simulink library "xbsIndex_r4"  (Simulink 7.1)
(part 7 of 9)

      mask init:
      | try
      |   tmp_gcb = gcb;
      |   tmp_gcbh = gcbh;
      |   if (strcmp('SysGenIndex',get_param(bdroot(tmp_gcbh),'tag')) && ~isempty(regexp(bdroot(tmp_gcb), '^xbs', 'once')))
      |     return;
      |   end;
      |   xlMungeMaskParams;
      |   block_config = 'sysgen:coregenimport_config';
      | 
      |   block_type='rs_decoder_v8_0';
      | 
      |   serialized_declarations = '{''aclken''=>''Bool'',''aresetn''=>''Bool'',''code_specification''=>''String'',''data_symbols''=>''Int'',''define_supported_r_in_values''=>''Bool'',''dsptool_ready''=>''Bool'',''erase''=>''Bool'',''error_statistics''=>''Bool'',''field_polynomial''=>''Int'',''generator_start''=>''Int'',''info''=>''Bool'',''ip_name''=>''String'',''ip_version''=>''String'',''ipcore_do_not_force_period''=>''Bool'',''ipcore_usecache''=>''Bool'',''ipcore_useipmodelcache''=>''Bool'',''marker_bits''=>''Bool'',''memory_style''=>''String'',''number_of_channels''=>''Int'',''number_of_marker_bits''=>''Int'',''number_of_puncture_patterns''=>''Int'',''number_of_supported_r_in_values''=>''Int'',''original_delayed_data''=>''Bool'',''output_check_symbols''=>''Bool'',''port_translation_map''=>''String'',''puncture_definition_file''=>''String'',''scaling_factor''=>''Int'',''self_recovering''=>''Bool'',''structural_sim''=>''Bool'',''supported_r_in_definition_file''=>''String'',''symbol_width''=>''String'',''symbols_per_block''=>''Int'',''trim_axipin_name''=>''Int'',''variable_block_length''=>''Bool'',''variable_number_of_check_symbols''=>''Bool'',''wrapper_available''=>''Bool'',''block_type''=>''String''}';
      |   ptable_ = xlblockprep(get_param(tmp_gcb, 'MaskWSVariables'));
      |   try
      |     xlBlockMoveCallback(tmp_gcbh);
      |   catch 
      |      clear global xl_updateicon_recursion_guard;
      |   end;
      | catch
      |   global dbgsysgen;
      |   if(~isempty(dbgsysgen) && dbgsysgen)
      |     e = regexprep(lasterr, '\n', '\nError: ');
      |     disp(['Error: While running MaskInit code on block ' tmp_gcb ': ' e]);
      |     error(e);
      |   end
      | end
      settings: CopyFcn=xlBlockMoveCallback(gcbh);  DeleteFcn=xlDestroyGui(gcbh);  ModelCloseFcn=xlDestroyGui(gcbh);  PreSaveFcn=xlBlockPreSaveCallback(gcbh);  PostSaveFcn=xlBlockPostSaveCallback(gcbh);  DestroyFcn=xlDestroyGui(gcbh);  OpenFcn=xlOpenGui(gcbh, 'rs_decoder_v8_0_gui.xml', @rs_decoder_v8_0_enablement, @rs_decoder_v8_0_action)  CloseFcn=xlDestroyGui(gcbh);  MoveFcn=xlBlockMoveCallback(gcbh);
      mask Help: eval('');xlDoc('-book','sysgen','-topic','Reed_Solomon_Decoder_8_0');
      mask StyleString: popup(Custom|DVB|ATSC|G.709|CCSDS|IESS-308(All)|IESS-308(126)|IESS-308(194)|IESS-308(208)|IESS-308(219)|IESS-308(225)|IEEE-802.16),popup(3|4|5|6|7|8|9|10|11|12),edit,edit,edit,edit,checkbox,edit,edit,edit,checkbox,edit,checkbox,edit,edit,edit,checkbox,popup(Automatic|Block|Distributed),edit,checkbox,edit,edit,edit,checkbox,edit,checkbox,edit,checkbox,edit,checkbox,edit,checkbox,edit,checkbox,edit,checkbox,edit,checkbox,edit,edit,edit,edit,edit,edit,edit,edit,edit,edit,edit,edit,edit,edit,edit,edit,edit
      mask Display:
      | fprintf('','COMMENT: begin icon graphics');
      | patch([0 0 2 2 ],[142 60 60 142 ],[5.650000e-001 6.550000e-001 5.500000e-001 ]);
      | patch([0 0 2 2 ],[52 30 30 52 ],[4.100000e-001 4.700000e-001 4.000000e-001 ]);
      | patch([0 0 2 2 ],[22 0 0 22 ],[2.550000e-001 2.850000e-001 2.500000e-001 ]);
      | patch([93 93 95 95 ],[125 117 117 125 ],[5.650000e-001 6.550000e-001 5.500000e-001 ]);
      | patch([93 93 95 95 ],[115 87 87 115 ],[4.100000e-001 4.700000e-001 4.000000e-001 ]);
      | patch([93 93 95 95 ],[85 47 47 85 ],[2.550000e-001 2.850000e-001 2.500000e-001 ]);
      | patch([93 93 95 95 ],[45 17 17 45 ],[7.200000e-001 8.400000e-001 7.000000e-001 ]);
      | patch([2 92 92 2 2 ],[0 0 142 142 0 ],[7.200000e-001 8.400000e-001 7.000000e-001 ]);
      | plot([2 92 92 2 2 ],[0 0 142 142 0 ]);
      | 
      | 
      | patch([18.075 36.86 49.86 62.86 75.86 49.86 31.075 18.075 ],[85.43 85.43 98.43 85.43 98.43 98.43 98.43 85.43 ],[1 1 1 ]);
      | patch([31.075 49.86 36.86 18.075 31.075 ],[72.43 72.43 85.43 85.43 72.43 ],[0.916 0.952 0.91 ]);
      | patch([18.075 36.86 49.86 31.075 18.075 ],[59.43 59.43 72.43 72.43 59.43 ],[1 1 1 ]);
      | patch([31.075 75.86 62.86 49.86 36.86 18.075 31.075 ],[46.43 46.43 59.43 46.43 59.43 59.43 46.43 ],[0.916 0.952 0.91 ]);
      | fprintf('','COMMENT: end icon graphics');
      | fprintf('','COMMENT: begin icon text');
      | color('black');port_label('input',1,'  input_tvalid  ');
      | color('black');port_label('input',2,'  input_tdata_data_in  ');
      | color('black');port_label('input',3,'  input_tlast  ');
      | color('black');port_label('input',4,'  output_tready  ');
      | color('black');port_label('input',5,'  stat_tready  ');
      | color('black');port_label('output',1,'  input_tready  ');
      | color('black');port_label('output',2,'  output_tvalid  ');
      | color('black');port_label('output',3,'  output_tdata_data_out  ');
      | color('black');port_label('output',4,'  output_tlast  ');
      | color('black');port_label('output',5,'  stat_tvalid  ');
      | color('black');port_label('output',6,'  stat_tdata_err_cnt  ');
      | color('black');port_label('output',7,'  stat_tdata_err_found  ');
      | color('black');port_label('output',8,'  stat_tdata_fail  ');
      | color('black');port_label('output',9,'  event_s_input_tlast_missing  ');
      | color('black');port_label('output',10,'  event_s_input_tlast_unexpected  ');
      | color('black');port_label('output',11,'  event_s_ctrl_tdata_invalid  ');
      | fprintf('','COMMENT: end icon text');
  "Reed-Solomon Encoder 6.1 " : S-Function  LoadFcn=xlBlockLoadCallback(gcbh);  FunctionName=sysgen  Parameters=ptable_  EnableBusSupport=off  mask(Xilinx Reed-Solomon Encoder 6.1 Block){infoedit=Reed-Solomon Encoder 6.1. The encoder transforms each block of k information symbols presented serially at the input port to a block of n symbols presented serially at the output port., code_specification_sgadvanced=, code_specification=Custom, number_of_channels=1, variable_number_of_check_symbols_sgadvanced=, variable_number_of_check_symbols=off, variable_block_length_sgadvanced=, variable_block_length=off, nd_sgadvanced=, nd=off, rdy_sgadvanced=, rdy=off, rfd_sgadvanced=, rfd=off, rffd_sgadvanced=, rffd=off, rst_sgadvanced=, rst=off, en_sgadvanced=, en=off, symbol_width_sgadvanced=, symbol_width=8, symbol_per_block=255, data_symbols=239, field_polynomial=0, generator_start=0, scaling_factor=1, memory_style_sgadvanced=, memory_style=Automatic, check_symbol_generator_sgadvanced=, check_symbol_generator=Fixed_Architecture, xl_use_area_sgadvanced=, xl_use_area=off, xl_area=[0,0,0,0,0,0,0], ip_name=Reed-Solomon Encoder, ip_version=6.1, has_advanced_control=0, sggui_pos=-1,-1,-1,-1, block_type=rs_encoder_v6_1, block_version=, sg_icon_stat=95,142,-1,-1,white,green,0,07734,right,,[ ],[ ], sg_mask_display=|, sg_list_contents=, sg_blockgui_xml=}
      mask sg_mask_display=|
      | fprintf('','COMMENT: begin icon graphics');
      | patch([0 95 95 0 0 ],[0 0 142 142 0 ],[0.72 0.84 0.7 ]);
      | plot([0 95 95 0 0 ],[0 0 142 142 0 ]);
      | patch([18.075 36.86 49.86 62.86 75.86 49.86 31.075 18.075 ],[85.43 85.43 98.43 85.43 98.43 98.43 98.43 85.43 ],[1 1 1 ]);
      | patch([31.075 49.86 36.86 18.075 31.075 ],[72.43 72.43 85.43 85.43 72.43 ],[0.916 0.952 0.91 ]);
      | patch([18.075 36.86 49.86 31.075 18.075 ],[59.43 59.43 72.43 72.43 59.43 ],[1 1 1 ]);
      | patch([31.075 75.86 62.86 49.86 36.86 18.075 31.075 ],[46.43 46.43 59.43 46.43 59.43 59.43 46.43 ],[0.916 0.952 0.91 ]);
      | fprintf('','COMMENT: end icon graphics');
      | fprintf('','COMMENT: begin icon text');
      | fprintf('','COMMENT: end icon text');
      mask prompts: infoedit ""; code_specification_sgadvanced ""; code_specification "Code specification (Predefined settings for popular standards)"; number_of_channels "Number of channels (Symbols for each channel are interlaced on DATA_IN and DATA_OUT)"; variable_number_of_check_symbols_sgadvanced ""; variable_number_of_check_symbols "Variable number of check symbols (Adds R_IN port)"; variable_block_length_sgadvanced ""; variable_block_length "Variable block length (Adds N_IN port)"; nd_sgadvanced ""; rdy_sgadvanced ""; rfd_sgadvanced ""; rffd_sgadvanced ""; rst_sgadvanced ""; en_sgadvanced ""; symbol_width_sgadvanced ""; symbol_width "Symbol width (Bus width of DATA_IN and DATA_OUT)"; symbol_per_block "Symbol per block (Total number of symbols in an encoded block, including check symbols)"; data_symbols "Data symbols (Number of original information symbols in block, prior to encoding)"; field_polynomial "Field polynomial (Galois Field primitive polynomial (enter in decimal))"; generator_start "Generator start (Galois Field logarithm of the first root of the Generator Polynomial)"; scaling_factor "Scaling factor (Scaling factor for Generator Polynomial root index)"; memory_style_sgadvanced ""; memory_style "Memory style (Force core to use this style of internal memory. 'Automatic' means let core decide)"; check_symbol_generator_sgadvanced ""; check_symbol_generator "Check symbol generator (Fixed architecture cannot be optimized)"; xl_use_area_sgadvanced ""; xl_use_area "Define FPGA area for resource estimation"; xl_area "FPGA area [slices, FFs, BRAMs, LUTs, IOBs, emb. mults, TBUFs]"; ip_name ""; ip_version ""; has_advanced_control ""; sggui_pos ""; block_type ""; block_version ""; sg_icon_stat ""; sg_mask_display ""; sg_list_contents ""; sg_blockgui_xml ""
      mask help: Reed-Solomon Encoder 6.1. The encoder transforms each block of k information symbols presented serially at the input port to a block of n symbols presented serially at the output port.
      mask init:
      | try
      |   tmp_gcb = gcb;
      |   tmp_gcbh = gcbh;
      |   if (strcmp('SysGenIndex',get_param(bdroot(tmp_gcbh),'tag')) && ~isempty(regexp(bdroot(tmp_gcb), '^xbs', 'once')))
      |     return;
      |   end;
      |   xlMungeMaskParams;
      |   block_config = 'sysgen_blockset:Removed_config';
      | 
      |   block_type='rs_encoder_v6_1';
      | nport = get_param(gcbh, 'ports');
      | nin = nport(1);
      | nout = nport(2);
      | 
      |   serialized_declarations = '{''check_symbol_generator''=>''String'',''code_specification''=>''String'',''data_symbols''=>''Int'',''en''=>''Bool'',''field_polynomial''=>''Int'',''generator_start''=>''Int'',''ip_name''=>''String'',''ip_version''=>''String'',''memory_style''=>''String'',''nd''=>''Bool'',''number_of_channels''=>''Int'',''rdy''=>''Bool'',''rfd''=>''Bool'',''rffd''=>''Bool'',''rst''=>''Bool'',''scaling_factor''=>''Int'',''symbol_per_block''=>''Int'',''symbol_width''=>''String'',''variable_block_length''=>''Bool'',''variable_number_of_check_symbols''=>''Bool'',''xl_use_area''=>''Bool'',''block_type''=>''String'',''nin''=>''Double'',''nout''=>''Double''}';
      |   ptable_ = xlblockprep(get_param(tmp_gcb, 'MaskWSVariables'));
      |   try
      |     xlBlockMoveCallback(tmp_gcbh);
      |   catch 
      |      clear global xl_updateicon_recursion_guard;
      |   end;
      | catch
      |   global dbgsysgen;
      |   if(~isempty(dbgsysgen) && dbgsysgen)
      |     e = regexprep(lasterr, '\n', '\nError: ');
      |     disp(['Error: While running MaskInit code on block ' tmp_gcb ': ' e]);
      |     error(e);
      |   end
      | end
      settings: CopyFcn=xlBlockMoveCallback(gcbh);  DeleteFcn=xlDestroyGui(gcbh);  ModelCloseFcn=xlDestroyGui(gcbh);  PreSaveFcn=xlBlockPreSaveCallback(gcbh);  PostSaveFcn=xlBlockPostSaveCallback(gcbh);  DestroyFcn=xlDestroyGui(gcbh);  OpenFcn=xlOpenGui(gcbh, 'rs_encoder_v6_1_gui.xml', @xlremovedenablement, -1)  CloseFcn=xlDestroyGui(gcbh);  MoveFcn=xlBlockMoveCallback(gcbh);
      mask Help: eval('');xlDoc('-book','sysgen','-topic','Reed_Solomon_Encoder_6_1');
      mask StyleString: edit,edit,popup(Custom|DVB|ATSC|CCSDS|ITU_J_83_Annex_B|IESS_308_126|IESS_308_194|IESS_308_208|IESS_308_219|IESS_308_225),edit,edit,checkbox,edit,checkbox,edit,checkbox,edit,checkbox,edit,checkbox,edit,checkbox,edit,checkbox,edit,checkbox,edit,popup(3|4|5|6|7|8|9|10|11|12),edit,edit,edit,edit,edit,edit,popup(Automatic|Block|Distributed),edit,popup(Fixed_Architecture|Optimized_For_Area|Optimized_For_Flexibility),edit,checkbox,edit,edit,edit,edit,edit,edit,edit,edit,edit,edit,edit
      mask Display:
      | fprintf('','COMMENT: begin icon graphics');
      | patch([0 95 95 0 0 ],[0 0 142 142 0 ],[0.72 0.84 0.7 ]);
      | plot([0 95 95 0 0 ],[0 0 142 142 0 ]);
      | patch([18.075 36.86 49.86 62.86 75.86 49.86 31.075 18.075 ],[85.43 85.43 98.43 85.43 98.43 98.43 98.43 85.43 ],[1 1 1 ]);
      | patch([31.075 49.86 36.86 18.075 31.075 ],[72.43 72.43 85.43 85.43 72.43 ],[0.916 0.952 0.91 ]);
      | patch([18.075 36.86 49.86 31.075 18.075 ],[59.43 59.43 72.43 72.43 59.43 ],[1 1 1 ]);
      | patch([31.075 75.86 62.86 49.86 36.86 18.075 31.075 ],[46.43 46.43 59.43 46.43 59.43 59.43 46.43 ],[0.916 0.952 0.91 ]);
      | fprintf('','COMMENT: end icon graphics');
      | fprintf('','COMMENT: begin icon text');
      | fprintf('','COMMENT: end icon text');
  "Reed-Solomon Encoder 7.0 " : S-Function  LoadFcn=xlBlockLoadCallback(gcbh);  FunctionName=sysgen  Parameters=ptable_  EnableBusSupport=off  mask(Xilinx Reed-Solomon Encoder 7.0  Block){code_specification=Custom, variable_number_of_check_symbols_sgadvanced=, variable_number_of_check_symbols=off, variable_block_length_sgadvanced=, variable_block_length=off, symbol_width=8, field_polynomial=0, scaling_factor=1, generator_start=0, symbol_per_block=255, data_symbols=239, check_symbol_generator_sgadvanced=, check_symbol_generator=Fixed_Architecture, memory_style=Automatic, number_of_channels=1, ce_sgadvanced=, ce=off, rdy_sgadvanced=, rdy=off, nd_sgadvanced=, nd=off, rfd_sgadvanced=, rfd=off, sclr_sgadvanced=, sclr=off, rffd_sgadvanced=, rffd=off, ip_name=Reed-Solomon Encoder, ip_version=7.0, dsptool_ready=false, ipcore_usecache=true, ipcore_useipmodelcache=true, wrapper_available=true, port_translation_map={ 'ce' => 'en', 'sclr' => 'rst'}, structural_sim=true, ipcore_do_not_force_period=true, has_advanced_control=0, sggui_pos=-1,-1,-1,-1, block_type=rs_encoder_v7_0, block_version=, sg_icon_stat=95,142,3,2,white,green,0,abcad2e4,right,,[ ],[ ], sg_mask_display=|, sg_list_contents=, sg_blockgui_xml=}
      mask sg_mask_display=|
      | fprintf('','COMMENT: begin icon graphics');
      | patch([0 95 95 0 0 ],[0 0 142 142 0 ],[0.72 0.84 0.7 ]);
      | plot([0 95 95 0 0 ],[0 0 142 142 0 ]);
      | patch([18.075 36.86 49.86 62.86 75.86 49.86 31.075 18.075 ],[85.43 85.43 98.43 85.43 98.43 98.43 98.43 85.43 ],[1 1 1 ]);
      | patch([31.075 49.86 36.86 18.075 31.075 ],[72.43 72.43 85.43 85.43 72.43 ],[0.916 0.952 0.91 ]);
      | patch([18.075 36.86 49.86 31.075 18.075 ],[59.43 59.43 72.43 72.43 59.43 ],[1 1 1 ]);
      | patch([31.075 75.86 62.86 49.86 36.86 18.075 31.075 ],[46.43 46.43 59.43 46.43 59.43 59.43 46.43 ],[0.916 0.952 0.91 ]);
      | fprintf('','COMMENT: end icon graphics');
      | fprintf('','COMMENT: begin icon text');
      | color('black');port_label('input',1,'data_in');
      | color('black');port_label('input',2,'bypass');
      | color('black');port_label('input',3,'start');
      | color('black');port_label('output',1,'data_out');
      | color('black');port_label('output',2,'info');
      | fprintf('','COMMENT: end icon text');
      mask prompts: code_specification "Code Specification"; variable_number_of_check_symbols_sgadvanced ""; variable_number_of_check_symbols "Variable Number Of Check Symbols (r)"; variable_block_length_sgadvanced ""; variable_block_length "Variable Block Length"; symbol_width "Symbol Width"; field_polynomial "Field Polynomial"; scaling_factor "Scaling Factor (h)"; generator_start "Generator Start"; symbol_per_block "Symbols Per Block (n)"; data_symbols "Data Symbols (k)"; check_symbol_generator_sgadvanced ""; check_symbol_generator ""; memory_style "Memory Style"; number_of_channels "Number Of Channels"; ce_sgadvanced ""; rdy_sgadvanced ""; nd_sgadvanced ""; rfd_sgadvanced ""; sclr_sgadvanced ""; rffd_sgadvanced ""; ip_name ""; ip_version ""; dsptool_ready ""; ipcore_usecache ""; ipcore_useipmodelcache ""; wrapper_available ""; port_translation_map ""; structural_sim ""; ipcore_do_not_force_period ""; has_advanced_control ""; sggui_pos ""; block_type ""; block_version ""; sg_icon_stat ""; sg_mask_display ""; sg_list_contents ""; sg_blockgui_xml ""
      mask help: Xilinx Reed-Solomon Encoder 7.0
      mask init:
      | try
      |   tmp_gcb = gcb;
      |   tmp_gcbh = gcbh;
      |   if (strcmp('SysGenIndex',get_param(bdroot(tmp_gcbh),'tag')) && ~isempty(regexp(bdroot(tmp_gcb), '^xbs', 'once')))
      |     return;
      |   end;
      |   xlMungeMaskParams;
      |   block_config = 'sysgen:coregenimport_config';
      | 
      |   block_type='rs_encoder_v7_0';
      | 
      |   serialized_declarations = '{''ce''=>''Bool'',''check_symbol_generator''=>''String'',''code_specification''=>''String'',''data_symbols''=>''Int'',''dsptool_ready''=>''Bool'',''field_polynomial''=>''Int'',''generator_start''=>''Int'',''ip_name''=>''String'',''ip_version''=>''String'',''ipcore_do_not_force_period''=>''Bool'',''ipcore_usecache''=>''Bool'',''ipcore_useipmodelcache''=>''Bool'',''memory_style''=>''String'',''nd''=>''Bool'',''number_of_channels''=>''Int'',''port_translation_map''=>''String'',''rdy''=>''Bool'',''rfd''=>''Bool'',''rffd''=>''Bool'',''scaling_factor''=>''Int'',''sclr''=>''Bool'',''structural_sim''=>''Bool'',''symbol_per_block''=>''Int'',''symbol_width''=>''String'',''variable_block_length''=>''Bool'',''variable_number_of_check_symbols''=>''Bool'',''wrapper_available''=>''Bool'',''block_type''=>''String''}';
      |   ptable_ = xlblockprep(get_param(tmp_gcb, 'MaskWSVariables'));
      |   try
      |     xlBlockMoveCallback(tmp_gcbh);
      |   catch 
      |      clear global xl_updateicon_recursion_guard;
      |   end;
      | catch
      |   global dbgsysgen;
      |   if(~isempty(dbgsysgen) && dbgsysgen)
      |     e = regexprep(lasterr, '\n', '\nError: ');
      |     disp(['Error: While running MaskInit code on block ' tmp_gcb ': ' e]);
      |     error(e);
      |   end
      | end
      settings: CopyFcn=xlBlockMoveCallback(gcbh);  DeleteFcn=xlDestroyGui(gcbh);  ModelCloseFcn=xlDestroyGui(gcbh);  PreSaveFcn=xlBlockPreSaveCallback(gcbh);  PostSaveFcn=xlBlockPostSaveCallback(gcbh);  DestroyFcn=xlDestroyGui(gcbh);  OpenFcn=xlOpenGui(gcbh, 'rs_encoder_v7_0_gui.xml', @xlipmagiccallback_pass_evaluate_params, @xlipmagicaction)  CloseFcn=xlDestroyGui(gcbh);  MoveFcn=xlBlockMoveCallback(gcbh);
      mask Help: eval('');xlDoc('-book','sysgen','-topic','Reed_Solomon_Encoder_7_0');
      mask StyleString: popup(Custom|DVB|ATSC|G_709|ETSI_BRAN|CCSDS|ITU_J_83_Annex_B|IESS_308_126|IESS_308_194|IESS_308_208|IESS_308_219|IESS_308_225),edit,checkbox,edit,checkbox,popup(3|4|5|6|7|8|9|10|11|12),edit,edit,edit,edit,edit,edit,popup(Fixed_Architecture|Optimized_For_Area|Optimized_For_Flexibility),popup(Automatic|Block|Distributed),edit,edit,checkbox,edit,checkbox,edit,checkbox,edit,checkbox,edit,checkbox,edit,checkbox,edit,edit,edit,edit,edit,edit,edit,edit,edit,edit,edit,edit,edit,edit,edit,edit,edit
      mask Display:
      | fprintf('','COMMENT: begin icon graphics');
      | patch([0 95 95 0 0 ],[0 0 142 142 0 ],[0.72 0.84 0.7 ]);
      | plot([0 95 95 0 0 ],[0 0 142 142 0 ]);
      | patch([18.075 36.86 49.86 62.86 75.86 49.86 31.075 18.075 ],[85.43 85.43 98.43 85.43 98.43 98.43 98.43 85.43 ],[1 1 1 ]);
      | patch([31.075 49.86 36.86 18.075 31.075 ],[72.43 72.43 85.43 85.43 72.43 ],[0.916 0.952 0.91 ]);
      | patch([18.075 36.86 49.86 31.075 18.075 ],[59.43 59.43 72.43 72.43 59.43 ],[1 1 1 ]);
      | patch([31.075 75.86 62.86 49.86 36.86 18.075 31.075 ],[46.43 46.43 59.43 46.43 59.43 59.43 46.43 ],[0.916 0.952 0.91 ]);
      | fprintf('','COMMENT: end icon graphics');
      | fprintf('','COMMENT: begin icon text');
      | color('black');port_label('input',1,'data_in');
      | color('black');port_label('input',2,'bypass');
      | color('black');port_label('input',3,'start');
      | color('black');port_label('output',1,'data_out');
      | color('black');port_label('output',2,'info');
      | fprintf('','COMMENT: end icon text');
  "Reed-Solomon Encoder 7.1 " : S-Function  LoadFcn=xlBlockLoadCallback(gcbh);  FunctionName=sysgen  Parameters=ptable_  EnableBusSupport=off  mask(Xilinx Reed-Solomon Encoder 7.1  Block){code_specification=Custom, variable_number_of_check_symbols_sgadvanced=, variable_number_of_check_symbols=off, variable_block_length_sgadvanced=, variable_block_length=off, symbol_width=8, field_polynomial=0, scaling_factor=1, generator_start=0, symbol_per_block=255, data_symbols=239, check_symbol_generator_sgadvanced=, check_symbol_generator=Fixed_Architecture, memory_style=Automatic, number_of_channels=1, ce_sgadvanced=, ce=off, rdy_sgadvanced=, rdy=off, nd_sgadvanced=, nd=off, rfd_sgadvanced=, rfd=off, sclr_sgadvanced=, sclr=off, rffd_sgadvanced=, rffd=off, ip_name=Reed-Solomon Encoder, ip_version=7.1, dsptool_ready=false, ipcore_usecache=true, ipcore_useipmodelcache=true, wrapper_available=true, port_translation_map={ 'ce' => 'en', 'sclr' => 'rst'}, structural_sim=false, ipcore_do_not_force_period=true, has_advanced_control=0, sggui_pos=-1,-1,-1,-1, block_type=rs_encoder_v7_1, block_version=, sg_icon_stat=95,142,3,2,white,green,0,abcad2e4,right,,[ ],[ ], sg_mask_display=|, sg_list_contents=, sg_blockgui_xml=}
      mask sg_mask_display=|
      | fprintf('','COMMENT: begin icon graphics');
      | patch([0 95 95 0 0 ],[0 0 142 142 0 ],[0.72 0.84 0.7 ]);
      | plot([0 95 95 0 0 ],[0 0 142 142 0 ]);
      | patch([18.075 36.86 49.86 62.86 75.86 49.86 31.075 18.075 ],[85.43 85.43 98.43 85.43 98.43 98.43 98.43 85.43 ],[1 1 1 ]);
      | patch([31.075 49.86 36.86 18.075 31.075 ],[72.43 72.43 85.43 85.43 72.43 ],[0.916 0.952 0.91 ]);
      | patch([18.075 36.86 49.86 31.075 18.075 ],[59.43 59.43 72.43 72.43 59.43 ],[1 1 1 ]);
      | patch([31.075 75.86 62.86 49.86 36.86 18.075 31.075 ],[46.43 46.43 59.43 46.43 59.43 59.43 46.43 ],[0.916 0.952 0.91 ]);
      | fprintf('','COMMENT: end icon graphics');
      | fprintf('','COMMENT: begin icon text');
      | color('black');port_label('input',1,'data_in');
      | color('black');port_label('input',2,'bypass');
      | color('black');port_label('input',3,'start');
      | color('black');port_label('output',1,'data_out');
      | color('black');port_label('output',2,'info');
      | fprintf('','COMMENT: end icon text');
      mask prompts: code_specification "Code Specification"; variable_number_of_check_symbols_sgadvanced ""; variable_number_of_check_symbols "Variable Number Of Check Symbols (r)"; variable_block_length_sgadvanced ""; variable_block_length "Variable Block Length"; symbol_width "Symbol Width"; field_polynomial "Field Polynomial"; scaling_factor "Scaling Factor (h)"; generator_start "Generator Start"; symbol_per_block "Symbols Per Block (n)"; data_symbols "Data Symbols (k)"; check_symbol_generator_sgadvanced ""; check_symbol_generator ""; memory_style "Memory Style"; number_of_channels "Number Of Channels"; ce_sgadvanced ""; rdy_sgadvanced ""; nd_sgadvanced ""; rfd_sgadvanced ""; sclr_sgadvanced ""; rffd_sgadvanced ""; ip_name ""; ip_version ""; dsptool_ready ""; ipcore_usecache ""; ipcore_useipmodelcache ""; wrapper_available ""; port_translation_map ""; structural_sim ""; ipcore_do_not_force_period ""; has_advanced_control ""; sggui_pos ""; block_type ""; block_version ""; sg_icon_stat ""; sg_mask_display ""; sg_list_contents ""; sg_blockgui_xml ""
      mask help: Xilinx Reed-Solomon Encoder 7.1
      mask init:
      | try
      |   tmp_gcb = gcb;
      |   tmp_gcbh = gcbh;
      |   if (strcmp('SysGenIndex',get_param(bdroot(tmp_gcbh),'tag')) && ~isempty(regexp(bdroot(tmp_gcb), '^xbs', 'once')))
      |     return;
      |   end;
      |   xlMungeMaskParams;
      |   block_config = 'sysgen:coregenimport_config';
      | 
      |   block_type='rs_encoder_v7_1';
      | 
      |   serialized_declarations = '{''ce''=>''Bool'',''check_symbol_generator''=>''String'',''code_specification''=>''String'',''data_symbols''=>''Int'',''dsptool_ready''=>''Bool'',''field_polynomial''=>''Int'',''generator_start''=>''Int'',''ip_name''=>''String'',''ip_version''=>''String'',''ipcore_do_not_force_period''=>''Bool'',''ipcore_usecache''=>''Bool'',''ipcore_useipmodelcache''=>''Bool'',''memory_style''=>''String'',''nd''=>''Bool'',''number_of_channels''=>''Int'',''port_translation_map''=>''String'',''rdy''=>''Bool'',''rfd''=>''Bool'',''rffd''=>''Bool'',''scaling_factor''=>''Int'',''sclr''=>''Bool'',''structural_sim''=>''Bool'',''symbol_per_block''=>''Int'',''symbol_width''=>''String'',''variable_block_length''=>''Bool'',''variable_number_of_check_symbols''=>''Bool'',''wrapper_available''=>''Bool'',''block_type''=>''String''}';
      |   ptable_ = xlblockprep(get_param(tmp_gcb, 'MaskWSVariables'));
      |   try
      |     xlBlockMoveCallback(tmp_gcbh);
      |   catch 
      |      clear global xl_updateicon_recursion_guard;
      |   end;
      | catch
      |   global dbgsysgen;
      |   if(~isempty(dbgsysgen) && dbgsysgen)
      |     e = regexprep(lasterr, '\n', '\nError: ');
      |     disp(['Error: While running MaskInit code on block ' tmp_gcb ': ' e]);
      |     error(e);
      |   end
      | end
      settings: CopyFcn=xlBlockMoveCallback(gcbh);  DeleteFcn=xlDestroyGui(gcbh);  ModelCloseFcn=xlDestroyGui(gcbh);  PreSaveFcn=xlBlockPreSaveCallback(gcbh);  PostSaveFcn=xlBlockPostSaveCallback(gcbh);  DestroyFcn=xlDestroyGui(gcbh);  OpenFcn=xlOpenGui(gcbh, 'rs_encoder_v7_1_gui.xml', @xlipmagiccallback_pass_evaluate_params, @xlipmagicaction)  CloseFcn=xlDestroyGui(gcbh);  MoveFcn=xlBlockMoveCallback(gcbh);
      mask Help: eval('');xlDoc('-book','sysgen','-topic','Reed_Solomon_Encoder_7_1');
      mask StyleString: popup(Custom|DVB|ATSC|G_709|ETSI_BRAN|CCSDS|ITU_J_83_Annex_B|IESS_308_126|IESS_308_194|IESS_308_208|IESS_308_219|IESS_308_225),edit,checkbox,edit,checkbox,popup(3|4|5|6|7|8|9|10|11|12),edit,edit,edit,edit,edit,edit,popup(Fixed_Architecture|Optimized_For_Area|Optimized_For_Flexibility),popup(Automatic|Block|Distributed),edit,edit,checkbox,edit,checkbox,edit,checkbox,edit,checkbox,edit,checkbox,edit,checkbox,edit,edit,edit,edit,edit,edit,edit,edit,edit,edit,edit,edit,edit,edit,edit,edit,edit
      mask Display:
      | fprintf('','COMMENT: begin icon graphics');
      | patch([0 95 95 0 0 ],[0 0 142 142 0 ],[0.72 0.84 0.7 ]);
      | plot([0 95 95 0 0 ],[0 0 142 142 0 ]);
      | patch([18.075 36.86 49.86 62.86 75.86 49.86 31.075 18.075 ],[85.43 85.43 98.43 85.43 98.43 98.43 98.43 85.43 ],[1 1 1 ]);
      | patch([31.075 49.86 36.86 18.075 31.075 ],[72.43 72.43 85.43 85.43 72.43 ],[0.916 0.952 0.91 ]);
      | patch([18.075 36.86 49.86 31.075 18.075 ],[59.43 59.43 72.43 72.43 59.43 ],[1 1 1 ]);
      | patch([31.075 75.86 62.86 49.86 36.86 18.075 31.075 ],[46.43 46.43 59.43 46.43 59.43 59.43 46.43 ],[0.916 0.952 0.91 ]);
      | fprintf('','COMMENT: end icon graphics');
      | fprintf('','COMMENT: begin icon text');
      | color('black');port_label('input',1,'data_in');
      | color('black');port_label('input',2,'bypass');
      | color('black');port_label('input',3,'start');
      | color('black');port_label('output',1,'data_out');
      | color('black');port_label('output',2,'info');
      | fprintf('','COMMENT: end icon text');
  "Reed-Solomon Encoder 8.0 " : S-Function  LoadFcn=xlBlockLoadCallback(gcbh);  FunctionName=sysgen  Parameters=ptable_  EnableBusSupport=off  mask(Xilinx Reed-Solomon Encoder 8.0  Block){code_specification=Custom, variable_number_of_check_symbols_sgadvanced=, variable_number_of_check_symbols=off, variable_block_length_sgadvanced=, variable_block_length=off, symbol_width=8, field_polynomial=0, scaling_factor=1, generator_start=0, symbol_per_block=255, data_symbols=239, check_symbol_generator_sgadvanced=, check_symbol_generator=Fixed_Architecture, memory_style=Automatic, number_of_channels=1, aclken_sgadvanced=, aclken=off, output_has_tready_sgadvanced=, output_has_tready=off, aresetn_sgadvanced=, aresetn=off, info_sgadvanced=, info=off, marker_bits_sgadvanced=, marker_bits=off, number_of_marker_bits=1, trim_axipin_name=on, ip_name=Reed-Solomon Encoder, ip_version=8.0, dsptool_ready=false, ipcore_usecache=true, ipcore_useipmodelcache=true, wrapper_available=true, port_translation_map={ 'aclken' => 'en', 'aresetn' => 'rst'}, structural_sim=false, ipcore_do_not_force_period=true, has_advanced_control=0, sggui_pos=-1,-1,-1,-1, block_type=rs_encoder_v8_0, block_version=, sg_icon_stat=215,223,3,6,white,green,0,414e65fd,right,,[2 2 2 ],[2 3 3 3 1 1 ], sg_mask_display=|, sg_list_contents=, sg_blockgui_xml=}
      mask sg_mask_display=|
      | fprintf('','COMMENT: begin icon graphics');
      | patch([0 0 4 4 ],[210 8 8 210 ],[5.133333e-001 5.933333e-001 5.000000e-001 ]);
      | patch([211 211 215 215 ],[211 187 187 211 ],[5.133333e-001 5.933333e-001 5.000000e-001 ]);
      | patch([211 211 215 215 ],[176 82 82 176 ],[3.066667e-001 3.466667e-001 3.000000e-001 ]);
      | patch([211 211 215 215 ],[71 12 12 71 ],[7.200000e-001 8.400000e-001 7.000000e-001 ]);
      | patch([4 210 210 4 4 ],[0 0 223 223 0 ],[7.200000e-001 8.400000e-001 7.000000e-001 ]);
      | plot([4 210 210 4 4 ],[0 0 223 223 0 ]);
      |
      |
      | patch([40.25 83.6 113.6 143.6 173.6 113.6 70.25 40.25 ],[144.3 144.3 174.3 144.3 174.3 174.3 174.3 144.3 ],[1 1 1 ]);
      | patch([70.25 113.6 83.6 40.25 70.25 ],[114.3 114.3 144.3 144.3 114.3 ],[0.916 0.952 0.91 ]);
      | patch([40.25 83.6 113.6 70.25 40.25 ],[84.3 84.3 114.3 114.3 84.3 ],[1 1 1 ]);
      | patch([70.25 173.6 143.6 113.6 83.6 40.25 70.25 ],[54.3 54.3 84.3 54.3 84.3 84.3 54.3 ],[0.916 0.952 0.91 ]);
      | fprintf('','COMMENT: end icon graphics');
      | fprintf('','COMMENT: begin icon text');
      | color('black');port_label('input',1,'  input_tvalid  ');
      | color('black');port_label('input',2,'  input_tdata_data_in  ');
      | color('black');port_label('input',3,'  input_tlast  ');
      | color('black');port_label('output',1,'  input_tready  ');
      | color('black');port_label('output',2,'  output_tvalid  ');
      | color('black');port_label('output',3,'  output_tdata_data_out  ');
      | color('black');port_label('output',4,'  output_tlast  ');
      | color('black');port_label('output',5,'  event_s_input_tlast_missing  ');
      | color('black');port_label('output',6,'  event_s_input_tlast_unexpected  ');
      | fprintf('','COMMENT: end icon text');
      mask prompts: code_specification "Code Specification"; variable_number_of_check_symbols_sgadvanced ""; variable_number_of_check_symbols "Variable Number Of Check Symbols (r)"; variable_block_length_sgadvanced ""; variable_block_length "Variable Block Length"; symbol_width "Symbol Width"; field_polynomial "Field Polynomial"; scaling_factor "Scaling Factor (h)"; generator_start "Generator Start"; symbol_per_block "Symbols Per Block (n)"; data_symbols "Data Symbols (k)"; check_symbol_generator_sgadvanced ""; check_symbol_generator ""; memory_style "Memory Style"; number_of_channels "Number Of Channels"; aclken_sgadvanced ""; output_has_tready_sgadvanced ""; output_has_tready "Output TREADY"; aresetn_sgadvanced ""; info_sgadvanced ""; info "Info bit"; marker_bits_sgadvanced ""; marker_bits "Marker Bits"; number_of_marker_bits "Number Of Marker Bits"; trim_axipin_name "Display shortened port names"; ip_name ""; ip_version ""; dsptool_ready ""; ipcore_usecache ""; ipcore_useipmodelcache ""; wrapper_available ""; port_translation_map ""; structural_sim ""; ipcore_do_not_force_period ""; has_advanced_control ""; sggui_pos ""; block_type ""; block_version ""; sg_icon_stat ""; sg_mask_display ""; sg_list_contents ""; sg_blockgui_xml ""
      mask help: Xilinx Reed-Solomon Encoder 8.0
      mask init:
      | try
      |   tmp_gcb = gcb;
      |   tmp_gcbh = gcbh;
      |   if (strcmp('SysGenIndex',get_param(bdroot(tmp_gcbh),'tag')) && ~isempty(regexp(bdroot(tmp_gcb), '^xbs', 'once')))
      |     return;
      |   end;
      |   xlMungeMaskParams;
      |   block_config = 'sysgen:coregenimport_config';
      | 
      |   block_type='rs_encoder_v8_0';
      | 
      |   serialized_declarations = '{''aclken''=>''Bool'',''aresetn''=>''Bool'',''check_symbol_generator''=>''String'',''code_specification''=>''String'',''data_symbols''=>''Int'',''dsptool_ready''=>''Bool'',''field_polynomial''=>''Int'',''generator_start''=>''Int'',''info''=>''Bool'',''ip_name''=>''String'',''ip_version''=>''String'',''ipcore_do_not_force_period''=>''Bool'',''ipcore_usecache''=>''Bool'',''ipcore_useipmodelcache''=>''Bool'',''marker_bits''=>''Bool'',''memory_style''=>''String'',''number_of_channels''=>''Int'',''number_of_marker_bits''=>''Int'',''output_has_tready''=>''Bool'',''port_translation_map''=>''String'',''scaling_factor''=>''Int'',''structural_sim''=>''Bool'',''symbol_per_block''=>''Int'',''symbol_width''=>''String'',''trim_axipin_name''=>''Int'',''variable_block_length''=>''Bool'',''variable_number_of_check_symbols''=>''Bool'',''wrapper_available''=>''Bool'',''block_type''=>''String''}';
      |   ptable_ = xlblockprep(get_param(tmp_gcb, 'MaskWSVariables'));
      |   try
      |     xlBlockMoveCallback(tmp_gcbh);
      |   catch 
      |      clear global xl_updateicon_recursion_guard;
      |   end;
      | catch
      |   global dbgsysgen;
      |   if(~isempty(dbgsysgen) && dbgsysgen)
      |     e = regexprep(lasterr, '\n', '\nError: ');
      |     disp(['Error: While running MaskInit code on block ' tmp_gcb ': ' e]);
      |     error(e);
      |   end
      | end
      settings: CopyFcn=xlBlockMoveCallback(gcbh);  DeleteFcn=xlDestroyGui(gcbh);  ModelCloseFcn=xlDestroyGui(gcbh);  PreSaveFcn=xlBlockPreSaveCallback(gcbh);  PostSaveFcn=xlBlockPostSaveCallback(gcbh);  DestroyFcn=xlDestroyGui(gcbh);  OpenFcn=xlOpenGui(gcbh, 'rs_encoder_v8_0_gui.xml', @xlipmagiccallback_pass_evaluate_params, @xlipmagicaction)  CloseFcn=xlDestroyGui(gcbh);  MoveFcn=xlBlockMoveCallback(gcbh);
      mask Help: eval('');xlDoc('-book','sysgen','-topic','Reed_Solomon_Encoder_8_0');
      mask StyleString: popup(Custom|DVB|ATSC|G_709|ETSI_BRAN|CCSDS|ITU_J_83_Annex_B|IESS_308_126|IESS_308_194|IESS_308_208|IESS_308_219|IESS_308_225),edit,checkbox,edit,checkbox,popup(3|4|5|6|7|8|9|10|11|12),edit,edit,edit,edit,edit,edit,popup(Fixed_Architecture|Optimized_For_Area|Optimized_For_Flexibility),popup(Automatic|Block|Distributed),edit,edit,checkbox,edit,checkbox,edit,checkbox,edit,checkbox,edit,checkbox,edit,checkbox,edit,edit,edit,edit,edit,edit,edit,edit,edit,edit,edit,edit,edit,edit,edit,edit,edit
      mask Display:
      | fprintf('','COMMENT: begin icon graphics');
      | patch([0 0 4 4 ],[210 8 8 210 ],[5.133333e-001 5.933333e-001 5.000000e-001 ]);
      | patch([211 211 215 215 ],[211 187 187 211 ],[5.133333e-001 5.933333e-001 5.000000e-001 ]);
      | patch([211 211 215 215 ],[176 82 82 176 ],[3.066667e-001 3.466667e-001 3.000000e-001 ]);
      | patch([211 211 215 215 ],[71 12 12 71 ],[7.200000e-001 8.400000e-001 7.000000e-001 ]);
      | patch([4 210 210 4 4 ],[0 0 223 223 0 ],[7.200000e-001 8.400000e-001 7.000000e-001 ]);
      | plot([4 210 210 4 4 ],[0 0 223 223 0 ]);
      | 
      | 
      | patch([40.25 83.6 113.6 143.6 173.6 113.6 70.25 40.25 ],[144.3 144.3 174.3 144.3 174.3 174.3 174.3 144.3 ],[1 1 1 ]);
      | patch([70.25 113.6 83.6 40.25 70.25 ],[114.3 114.3 144.3 144.3 114.3 ],[0.916 0.952 0.91 ]);
      | patch([40.25 83.6 113.6 70.25 40.25 ],[84.3 84.3 114.3 114.3 84.3 ],[1 1 1 ]);
      | patch([70.25 173.6 143.6 113.6 83.6 40.25 70.25 ],[54.3 54.3 84.3 54.3 84.3 84.3 54.3 ],[0.916 0.952 0.91 ]);
      | fprintf('','COMMENT: end icon graphics');
      | fprintf('','COMMENT: begin icon text');
      | color('black');port_label('input',1,'  input_tvalid  ');
      | color('black');port_label('input',2,'  input_tdata_data_in  ');
      | color('black');port_label('input',3,'  input_tlast  ');
      | color('black');port_label('output',1,'  input_tready  ');
      | color('black');port_label('output',2,'  output_tvalid  ');
      | color('black');port_label('output',3,'  output_tdata_data_out  ');
      | color('black');port_label('output',4,'  output_tlast  ');
      | color('black');port_label('output',5,'  event_s_input_tlast_missing  ');
      | color('black');port_label('output',6,'  event_s_input_tlast_unexpected  ');
      | fprintf('','COMMENT: end icon text');
  Register : S-Function  LoadFcn=xlBlockLoadCallback(gcbh);  FunctionName=sysgen  Parameters=ptable_  EnableBusSupport=off  mask(Xilinx Register Block){init=0, rst_sgadvanced=, rst=off, en_sgadvanced=, en=off, dbl_ovrd_sgadvanced=, dbl_ovrd=off, xl_use_area_sgadvanced=, xl_use_area=off, xl_area=[0,0,0,0,0,0,0], has_advanced_control=0, sggui_pos=-1,-1,-1,-1, block_type=register, block_version=, sg_icon_stat=60,56,1,1,white,blue,0,c80657c5,right,,[ ],[ ], sg_mask_display=|, sg_list_contents=, sg_blockgui_xml=}
      mask sg_mask_display=|
      | fprintf('','COMMENT: begin icon graphics');
      | patch([0 60 60 0 0 ],[0 0 56 56 0 ],[0.77 0.82 0.91 ]);
      | plot([0 60 60 0 0 ],[0 0 56 56 0 ]);
      | patch([12.2 23.76 31.76 39.76 47.76 31.76 20.2 12.2 ],[36.88 36.88 44.88 36.88 44.88 44.88 44.88 36.88 ],[1 1 1 ]);
      | patch([20.2 31.76 23.76 12.2 20.2 ],[28.88 28.88 36.88 36.88 28.88 ],[0.931 0.946 0.973 ]);
      | patch([12.2 23.76 31.76 20.2 12.2 ],[20.88 20.88 28.88 28.88 20.88 ],[1 1 1 ]);
      | patch([20.2 47.76 39.76 31.76 23.76 12.2 20.2 ],[12.88 12.88 20.88 12.88 20.88 20.88 12.88 ],[0.931 0.946 0.973 ]);
      | fprintf('','COMMENT: end icon graphics');
      | fprintf('','COMMENT: begin icon text');
      | color('black');port_label('input',1,'d');
      | color('black');port_label('output',1,'q');
      | color('black');disp('z^{-1}','texmode','on');
      | fprintf('','COMMENT: end icon text');
      mask prompts: init "Initial value"; rst_sgadvanced ""; rst "Provide synchronous reset port"; en_sgadvanced ""; en "Provide enable port"; dbl_ovrd_sgadvanced ""; dbl_ovrd "Override with doubles"; xl_use_area_sgadvanced ""; xl_use_area "Define FPGA area for resource estimation"; xl_area "FPGA area [slices, FFs, BRAMs, LUTs, IOBs, emb. mults, TBUFs]"; has_advanced_control ""; sggui_pos ""; block_type ""; block_version ""; sg_icon_stat ""; sg_mask_display ""; sg_list_contents ""; sg_blockgui_xml ""
      mask help: Xilinx Register
      mask init:
      | try
      |   tmp_gcb = gcb;
      |   tmp_gcbh = gcbh;
      |   if (strcmp('SysGenIndex',get_param(bdroot(tmp_gcbh),'tag')) && ~isempty(regexp(bdroot(tmp_gcb), '^xbs', 'once')))
      |     return;
      |   end;
      |   xlMungeMaskParams;
      |   block_config = 'sysgen_blockset:Register_config';
      | 
      |   block_type='register';
      | 
      |   serialized_declarations = '{''dbl_ovrd''=>''Int'',''en''=>''Int'',''init''=>''Double'',''rst''=>''Int'',''block_type''=>''String''}';
      |   xlregister_init();
      |   ptable_ = xlblockprep(get_param(tmp_gcb, 'MaskWSVariables'));
      |   try
      |     xlBlockMoveCallback(tmp_gcbh);
      |   catch 
      |      clear global xl_updateicon_recursion_guard;
      |   end;
      | catch
      |   global dbgsysgen;
      |   if(~isempty(dbgsysgen) && dbgsysgen)
      |     e = regexprep(lasterr, '\n', '\nError: ');
      |     disp(['Error: While running MaskInit code on block ' tmp_gcb ': ' e]);
      |     error(e);
      |   end
      | end
      settings: CopyFcn=xlBlockMoveCallback(gcbh);  DeleteFcn=xlDestroyGui(gcbh);  ModelCloseFcn=xlDestroyGui(gcbh);  PreSaveFcn=xlBlockPreSaveCallback(gcbh);  PostSaveFcn=xlBlockPostSaveCallback(gcbh);  DestroyFcn=xlDestroyGui(gcbh);  OpenFcn=xlOpenGui(gcbh, 'register_gui.xml', @xlmagicenablement, -1)  CloseFcn=xlDestroyGui(gcbh);  MoveFcn=xlBlockMoveCallback(gcbh);
      mask Help: eval('');xlDoc('-book','sysgen','-topic','Register');
      mask Display:
      | fprintf('','COMMENT: begin icon graphics');
      | patch([0 60 60 0 0 ],[0 0 56 56 0 ],[0.77 0.82 0.91 ]);
      | plot([0 60 60 0 0 ],[0 0 56 56 0 ]);
      | patch([12.2 23.76 31.76 39.76 47.76 31.76 20.2 12.2 ],[36.88 36.88 44.88 36.88 44.88 44.88 44.88 36.88 ],[1 1 1 ]);
      | patch([20.2 31.76 23.76 12.2 20.2 ],[28.88 28.88 36.88 36.88 28.88 ],[0.931 0.946 0.973 ]);
      | patch([12.2 23.76 31.76 20.2 12.2 ],[20.88 20.88 28.88 28.88 20.88 ],[1 1 1 ]);
      | patch([20.2 47.76 39.76 31.76 23.76 12.2 20.2 ],[12.88 12.88 20.88 12.88 20.88 20.88 12.88 ],[0.931 0.946 0.973 ]);
      | fprintf('','COMMENT: end icon graphics');
      | fprintf('','COMMENT: begin icon text');
      | color('black');port_label('input',1,'d');
      | color('black');port_label('output',1,'q');
      | color('black');disp('z^{-1}','texmode','on');
      | fprintf('','COMMENT: end icon text');
  Reinterpret : S-Function  LoadFcn=xlBlockLoadCallback(gcbh);  FunctionName=sysgen  Parameters=ptable_  EnableBusSupport=off  mask(Xilinx Type Reinterpreter Block){infoedit=Changes signal type without altering the binary representation.   You can change the signal between signed and unsigned, and relocate the binary point.<br><br>Hardware notes: In hardware this block costs nothing.<br><br>Example:  Suppose the input is 6 bits wide, signed, with 2 fractional bits, and the output is forced to unsigned with 0 fractional bits.  Then an input of -2.0 (1110.00 in binary 2's complement) becomes an output of 56 (111000 in binary)., force_arith_type_sgadvanced=, force_arith_type=off, arith_type_sgadvanced=, arith_type=Unsigned, force_bin_pt_sgadvanced=, force_bin_pt=off, bin_pt=0, has_advanced_control=0, sggui_pos=-1,-1,-1,-1, block_type=reinterpret, block_version=, sg_icon_stat=50,32,1,1,white,blue,0,6b04d0b0,right,,[ ],[ ], sg_mask_display=|, sg_list_contents=, sg_blockgui_xml=}
      mask sg_mask_display=|
      | fprintf('','COMMENT: begin icon graphics');
      | patch([0 50 50 0 0 ],[0 0 32 32 0 ],[0.77 0.82 0.91 ]);
      | plot([0 50 50 0 0 ],[0 0 32 32 0 ]);
      | patch([16.1 21.88 25.88 29.88 33.88 25.88 20.1 16.1 ],[20.44 20.44 24.44 20.44 24.44 24.44 24.44 20.44 ],[1 1 1 ]);
      | patch([20.1 25.88 21.88 16.1 20.1 ],[16.44 16.44 20.44 20.44 16.44 ],[0.931 0.946 0.973 ]);
      | patch([16.1 21.88 25.88 20.1 16.1 ],[12.44 12.44 16.44 16.44 12.44 ],[1 1 1 ]);
      | patch([20.1 33.88 29.88 25.88 21.88 16.1 20.1 ],[8.44 8.44 12.44 8.44 12.44 12.44 8.44 ],[0.931 0.946 0.973 ]);
      | fprintf('','COMMENT: end icon graphics');
      | fprintf('','COMMENT: begin icon text');
      |
      |
      | color('black');disp('reinterpret');
      | fprintf('','COMMENT: end icon text');
      mask prompts: infoedit ""; force_arith_type_sgadvanced ""; force_arith_type "Force Arithmetic Type"; arith_type_sgadvanced ""; arith_type "Output Arithmetic Type"; force_bin_pt_sgadvanced ""; force_bin_pt "Force Binary Point"; bin_pt "Output Binary Point"; has_advanced_control ""; sggui_pos ""; block_type ""; block_version ""; sg_icon_stat ""; sg_mask_display ""; sg_list_contents ""; sg_blockgui_xml ""
      mask help:
      | Changes signal type without altering the binary representation.   You can change the signal between signed and unsigned, and relocate the binary point.
      |
      | Hardware notes: In hardware this block costs nothing.
      |
      | Example:  Suppose the input is 6 bits wide, signed, with 2 fractional bits, and the output is forced to unsigned with 0 fractional bits.  Then an input of -2.0 (1110.00 in binary 2's complement) becomes an output of 56 (111000 in binary).
      mask init:
      | try
      |   tmp_gcb = gcb;
      |   tmp_gcbh = gcbh;
      |   if (strcmp('SysGenIndex',get_param(bdroot(tmp_gcbh),'tag')) && ~isempty(regexp(bdroot(tmp_gcb), '^xbs', 'once')))
      |     return;
      |   end;
      |   xlMungeMaskParams;
      |   block_config = 'sysgen_blockset:Reinterpret_config';
      | 
      |   block_type='reinterpret';
      | 
      |   serialized_declarations = '{''arith_type''=>''Int'',''bin_pt''=>''Int'',''force_arith_type''=>''Bool'',''force_bin_pt''=>''Bool'',''block_type''=>''String''}';
      |   ptable_ = xlblockprep(get_param(tmp_gcb, 'MaskWSVariables'));
      |   try
      |     xlBlockMoveCallback(tmp_gcbh);
      |   catch 
      |      clear global xl_updateicon_recursion_guard;
      |   end;
      | catch
      |   global dbgsysgen;
      |   if(~isempty(dbgsysgen) && dbgsysgen)
      |     e = regexprep(lasterr, '\n', '\nError: ');
      |     disp(['Error: While running MaskInit code on block ' tmp_gcb ': ' e]);
      |     error(e);
      |   end
      | end
      settings: CopyFcn=xlBlockMoveCallback(gcbh);  DeleteFcn=xlDestroyGui(gcbh);  ModelCloseFcn=xlDestroyGui(gcbh);  PreSaveFcn=xlBlockPreSaveCallback(gcbh);  PostSaveFcn=xlBlockPostSaveCallback(gcbh);  DestroyFcn=xlDestroyGui(gcbh);  OpenFcn=xlOpenGui(gcbh, 'reinterpret_gui.xml', @reinterpretenablement, -1)  CloseFcn=xlDestroyGui(gcbh);  MoveFcn=xlBlockMoveCallback(gcbh);
      mask Help: eval('');xlDoc('-book','sysgen','-topic','Reinterpret');
      mask StyleString: edit,edit,checkbox,edit,popup(Unsigned|Signed  (2's comp)|Floating-point),edit,checkbox,edit,edit,edit,edit,edit,edit,edit,edit,edit
      mask Display:
      | fprintf('','COMMENT: begin icon graphics');
      | patch([0 50 50 0 0 ],[0 0 32 32 0 ],[0.77 0.82 0.91 ]);
      | plot([0 50 50 0 0 ],[0 0 32 32 0 ]);
      | patch([16.1 21.88 25.88 29.88 33.88 25.88 20.1 16.1 ],[20.44 20.44 24.44 20.44 24.44 24.44 24.44 20.44 ],[1 1 1 ]);
      | patch([20.1 25.88 21.88 16.1 20.1 ],[16.44 16.44 20.44 20.44 16.44 ],[0.931 0.946 0.973 ]);
      | patch([16.1 21.88 25.88 20.1 16.1 ],[12.44 12.44 16.44 16.44 12.44 ],[1 1 1 ]);
      | patch([20.1 33.88 29.88 25.88 21.88 16.1 20.1 ],[8.44 8.44 12.44 8.44 12.44 12.44 8.44 ],[0.931 0.946 0.973 ]);
      | fprintf('','COMMENT: end icon graphics');
      | fprintf('','COMMENT: begin icon text');
      | 
      | 
      | color('black');disp('reinterpret');
      | fprintf('','COMMENT: end icon text');
  Relational : S-Function  LoadFcn=xlBlockLoadCallback(gcbh);  FunctionName=sysgen  Parameters=ptable_  EnableBusSupport=off  mask(Xilinx Arithmetic Relational Operator Block){mode_sgadvanced=, mode=a=b, en_sgadvanced=, en=off, latency=0, dbl_ovrd_sgadvanced=, dbl_ovrd=off, xl_use_area_sgadvanced=, xl_use_area=off, xl_area=[0,0,0,0,0,0,0], has_advanced_control=0, sggui_pos=-1,-1,-1,-1, block_type=relational, block_version=, sg_icon_stat=55,56,2,1,white,blue,0,2a81ff49,right,,[ ],[ ], sg_mask_display=|, sg_list_contents=, sg_blockgui_xml=}
      mask sg_mask_display=|
      | fprintf('','COMMENT: begin icon graphics');
      | patch([0 55 55 0 0 ],[0 0 56 56 0 ],[0.77 0.82 0.91 ]);
      | plot([0 55 55 0 0 ],[0 0 56 56 0 ]);
      | patch([11.425 21.54 28.54 35.54 42.54 28.54 18.425 11.425 ],[35.77 35.77 42.77 35.77 42.77 42.77 42.77 35.77 ],[1 1 1 ]);
      | patch([18.425 28.54 21.54 11.425 18.425 ],[28.77 28.77 35.77 35.77 28.77 ],[0.931 0.946 0.973 ]);
      | patch([11.425 21.54 28.54 18.425 11.425 ],[21.77 21.77 28.77 28.77 21.77 ],[1 1 1 ]);
      | patch([18.425 42.54 35.54 28.54 21.54 11.425 18.425 ],[14.77 14.77 21.77 14.77 21.77 21.77 14.77 ],[0.931 0.946 0.973 ]);
      | fprintf('','COMMENT: end icon graphics');
      | fprintf('','COMMENT: begin icon text');
      | color('black');port_label('input',1,'a');
      | color('black');port_label('input',2,'b');
      | color('black');port_label('output',1,'\bfa = b','texmode','on');
      | color('black');disp(' ');
      | fprintf('','COMMENT: end icon text');
      mask prompts: mode_sgadvanced ""; mode "Comparison:"; en_sgadvanced ""; en "Provide enable port"; dbl_ovrd_sgadvanced ""; dbl_ovrd "Override with doubles"; xl_use_area_sgadvanced ""; xl_use_area "Define FPGA area for resource estimation"; xl_area "FPGA area [slices, FFs, BRAMs, LUTs, IOBs, emb. mults, TBUFs]"; has_advanced_control ""; sggui_pos ""; block_type ""; block_version ""; sg_icon_stat ""; sg_mask_display ""; sg_list_contents ""; sg_blockgui_xml ""
      mask help: Xilinx Arithmetic Relational Operator
      mask init:
      | try
      |   tmp_gcb = gcb;
      |   tmp_gcbh = gcbh;
      |   if (strcmp('SysGenIndex',get_param(bdroot(tmp_gcbh),'tag')) && ~isempty(regexp(bdroot(tmp_gcb), '^xbs', 'once')))
      |     return;
      |   end;
      |   xlMungeMaskParams;
      |   block_config = 'sysgen_blockset:Relational_config';
      | 
      |   block_type='relational';
      | 
      |   serialized_declarations = '{''dbl_ovrd''=>''Int'',''en''=>''Int'',''latency''=>''Int'',''mode''=>''Int'',''block_type''=>''String''}';
      |   ptable_ = xlblockprep(get_param(tmp_gcb, 'MaskWSVariables'));
      |   try
      |     xlBlockMoveCallback(tmp_gcbh);
      |   catch 
      |      clear global xl_updateicon_recursion_guard;
      |   end;
      | catch
      |   global dbgsysgen;
      |   if(~isempty(dbgsysgen) && dbgsysgen)
      |     e = regexprep(lasterr, '\n', '\nError: ');
      |     disp(['Error: While running MaskInit code on block ' tmp_gcb ': ' e]);
      |     error(e);
      |   end
      | end
      settings: CopyFcn=xlBlockMoveCallback(gcbh);  DeleteFcn=xlDestroyGui(gcbh);  ModelCloseFcn=xlDestroyGui(gcbh);  PreSaveFcn=xlBlockPreSaveCallback(gcbh);  PostSaveFcn=xlBlockPostSaveCallback(gcbh);  DestroyFcn=xlDestroyGui(gcbh);  OpenFcn=xlOpenGui(gcbh, 'relational_gui.xml', @xlmagicenablement, -1)  CloseFcn=xlDestroyGui(gcbh);  MoveFcn=xlBlockMoveCallback(gcbh);
      mask Help: eval('');xlDoc('-book','sysgen','-topic','Relational');
      mask StyleString: edit,popup(a=b|a!=b|a<b|a>b|a<=b|a>=b),edit,checkbox,edit,edit,checkbox,edit,checkbox,edit,edit,edit,edit,edit,edit,edit,edit,edit
      mask Display:
      | fprintf('','COMMENT: begin icon graphics');
      | patch([0 55 55 0 0 ],[0 0 56 56 0 ],[0.77 0.82 0.91 ]);
      | plot([0 55 55 0 0 ],[0 0 56 56 0 ]);
      | patch([11.425 21.54 28.54 35.54 42.54 28.54 18.425 11.425 ],[35.77 35.77 42.77 35.77 42.77 42.77 42.77 35.77 ],[1 1 1 ]);
      | patch([18.425 28.54 21.54 11.425 18.425 ],[28.77 28.77 35.77 35.77 28.77 ],[0.931 0.946 0.973 ]);
      | patch([11.425 21.54 28.54 18.425 11.425 ],[21.77 21.77 28.77 28.77 21.77 ],[1 1 1 ]);
      | patch([18.425 42.54 35.54 28.54 21.54 11.425 18.425 ],[14.77 14.77 21.77 14.77 21.77 21.77 14.77 ],[0.931 0.946 0.973 ]);
      | fprintf('','COMMENT: end icon graphics');
      | fprintf('','COMMENT: begin icon text');
      | color('black');port_label('input',1,'a');
      | color('black');port_label('input',2,'b');
      | color('black');port_label('output',1,'\bfa = b','texmode','on');
      | color('black');disp(' ');
      | fprintf('','COMMENT: end icon text');
  Reset Generator : Subsystem  LoadFcn=xlBlockLoadCallback(gcbh);  mask(Xilinx Reset Generator Block){infoedit=Captures the user's reset signal that is running at the system sample rate, and produces a downsampled reset signal running at the rates specified on the block.  The downsampled reset signals are synchronized in the same way as they are during startup.  The RDY output signal indicates when the downsampled resets are no longer asserted after the input reset is detected., rates=[2 5], previous_rates=2  5, has_advanced_control=0, sggui_pos=-1,-1,-1,-1, block_type=resetgenerator, block_version=1.0, sg_icon_stat=55,52,1,3,white,blue,0,382607966eaa212ad1ba7a6776605633,right,,[ ],[ ], sg_mask_display=|, sg_list_contents=, sg_blockgui_xml=}
      mask sg_mask_display=|
      | fprintf('','COMMENT: begin icon graphics');
      | patch([0 55 55 0 0 ],[0 0 52 52 0 ],[0.77 0.82 0.91 ]);
      | plot([0 55 55 0 0 ],[0 0 52 52 0 ]);
      | patch([11.425 21.54 28.54 35.54 42.54 28.54 18.425 11.425 ],[33.77 33.77 40.77 33.77 40.77 40.77 40.77 33.77 ],[1 1 1 ]);
      | patch([18.425 28.54 21.54 11.425 18.425 ],[26.77 26.77 33.77 33.77 26.77 ],[0.931 0.946 0.973 ]);
      | patch([11.425 21.54 28.54 18.425 11.425 ],[19.77 19.77 26.77 26.77 19.77 ],[1 1 1 ]);
      | patch([18.425 42.54 35.54 28.54 21.54 11.425 18.425 ],[12.77 12.77 19.77 12.77 19.77 19.77 12.77 ],[0.931 0.946 0.973 ]);
      | fprintf('','COMMENT: end icon graphics');
      | fprintf('','COMMENT: begin icon text');
      | color('black');port_label('input',1,'rst');
      | color('black');port_label('output',1,'rst5');
      | color('black');port_label('output',2,'rst2');
      | color('black');port_label('output',3,'rdy');
      | fprintf('','COMMENT: end icon text');
      mask prompts: infoedit ""; rates "Specify design sample rates in MATLAB vector format, e.g. [2  4 16]"; previous_rates ""; has_advanced_control ""; sggui_pos ""; block_type ""; block_version ""; sg_icon_stat ""; sg_mask_display ""; sg_list_contents ""; sg_blockgui_xml ""
      mask help: Captures the user's reset signal that is running at the system sample rate, and produces a downsampled reset signal running at the rates specified on the block. The downsampled reset signals are synchronized in the same way as they are during startup. The RDY output signal indicates when the downsampled resets are no longer asserted after the input reset is detected.
      mask init:
      | try
      |   tmp_gcb = gcb;
      |   tmp_gcbh = gcbh;
      |   if (strcmp('SysGenIndex',get_param(bdroot(tmp_gcbh),'tag')) && ~isempty(regexp(bdroot(tmp_gcb), '^xbs', 'once')))
      |     return;
      |   end;
      |   xlMungeMaskParams;
      | 
      |   block_type='resetgenerator';
      | 
      |   serialized_declarations = '{''block_type''=>''String''}';
      |   xlReset_init();
      |   ptable_ = xlblockprep(get_param(tmp_gcb, 'MaskWSVariables'));
      |   try
      |     xlBlockMoveCallback(tmp_gcbh);
      |   catch 
      |      clear global xl_updateicon_recursion_guard;
      |   end;
      | catch
      |   global dbgsysgen;
      |   if(~isempty(dbgsysgen) && dbgsysgen)
      |     e = regexprep(lasterr, '\n', '\nError: ');
      |     disp(['Error: While running MaskInit code on block ' tmp_gcb ': ' e]);
      |     error(e);
      |   end
      | end
      settings: CopyFcn=tmp_gcbh = gcbh;set_param(tmp_gcbh,'linkstatus','none');xlBlockMoveCallback(gcbh);  DeleteFcn=xlDestroyGui(gcbh);  ModelCloseFcn=xlDestroyGui(gcbh);  PreSaveFcn=xlBlockPreSaveCallback(gcbh);  PostSaveFcn=xlBlockPostSaveCallback(gcbh);  DestroyFcn=xlDestroyGui(gcbh);  OpenFcn=xlOpenGui(gcbh, 'xlReset_gui.xml', -1, -1)  CloseFcn=xlDestroyGui(gcbh);  MoveFcn=xlBlockMoveCallback(gcbh);
      mask Help: eval('');xlDoc('-book','sysgen','-topic','Reset_Generator');
      mask Display:
      | fprintf('','COMMENT: begin icon graphics');
      | patch([0 55 55 0 0 ],[0 0 52 52 0 ],[0.77 0.82 0.91 ]);
      | plot([0 55 55 0 0 ],[0 0 52 52 0 ]);
      | patch([11.425 21.54 28.54 35.54 42.54 28.54 18.425 11.425 ],[33.77 33.77 40.77 33.77 40.77 40.77 40.77 33.77 ],[1 1 1 ]);
      | patch([18.425 28.54 21.54 11.425 18.425 ],[26.77 26.77 33.77 33.77 26.77 ],[0.931 0.946 0.973 ]);
      | patch([11.425 21.54 28.54 18.425 11.425 ],[19.77 19.77 26.77 26.77 19.77 ],[1 1 1 ]);
      | patch([18.425 42.54 35.54 28.54 21.54 11.425 18.425 ],[12.77 12.77 19.77 12.77 19.77 19.77 12.77 ],[0.931 0.946 0.973 ]);
      | fprintf('','COMMENT: end icon graphics');
      | fprintf('','COMMENT: begin icon text');
      | color('black');port_label('input',1,'rst');
      | color('black');port_label('output',1,'rst5');
      | color('black');port_label('output',2,'rst2');
      | color('black');port_label('output',3,'rdy');
      | fprintf('','COMMENT: end icon text');
  Resource Estimator : S-Function  Tag=resEstTag  LoadFcn=xlBlockLoadCallback(gcbh);  FunctionName=xlpermissive  Parameters=''  EnableBusSupport=off  mask(Xilinx Resource Estimator Block){Slices=0, FFs=0, BRAMs=0, LUTs=0, IOBs=0, EBMs=0, TBUFs=0, xl_use_estimator_area_sgadvanced=, xl_use_estimator_area=off, est_options_sgadvanced=, est_options=Estimate, xl_estimator_area=, mrp_directory=, simulink_period=, ShowPortLabels=, has_advanced_control=0, sggui_pos=-1,-1,-1,-1, block_type=resource_estimator, block_version=, sg_icon_stat=53,53,-1,-1,blue,white,0,07734,right,,[ ],[ ], sg_mask_display=|, sg_list_contents=, sg_blockgui_xml=}
      mask sg_mask_display=|
      | fprintf('','COMMENT: begin icon graphics');
      | patch([0 53 53 0 0 ],[0 0 53 53 0 ],[1 1 1 ]);
      | plot([0 53 53 0 0 ],[0 0 53 53 0 ]);
      | patch([10.425 20.54 27.54 34.54 41.54 27.54 17.425 10.425 ],[33.77 33.77 40.77 33.77 40.77 40.77 40.77 33.77 ],[0.839 0.874 0.937 ]);
      | patch([17.425 27.54 20.54 10.425 17.425 ],[26.77 26.77 33.77 33.77 26.77 ],[0.77 0.82 0.91 ]);
      | patch([10.425 20.54 27.54 17.425 10.425 ],[19.77 19.77 26.77 26.77 19.77 ],[0.839 0.874 0.937 ]);
      | patch([17.425 41.54 34.54 27.54 20.54 10.425 17.425 ],[12.77 12.77 19.77 12.77 19.77 19.77 12.77 ],[0.77 0.82 0.91 ]);
      | fprintf('','COMMENT: end icon graphics');
      | fprintf('','COMMENT: begin icon text');
      | fprintf('','COMMENT: end icon text');
      mask prompts: EBMs "Mults/DSP48s"; xl_use_estimator_area_sgadvanced ""; xl_use_estimator_area "Use area above"; est_options_sgadvanced ""; est_options "Estimate options"; xl_estimator_area ""; mrp_directory ""; simulink_period ""; ShowPortLabels ""; has_advanced_control ""; sggui_pos ""; block_type ""; block_version ""; sg_icon_stat ""; sg_mask_display ""; sg_list_contents ""; sg_blockgui_xml ""
      mask help: Xilinx Resource Estimator
      mask init:
      | try
      |   tmp_gcb = gcb;
      |   tmp_gcbh = gcbh;
      |   if (strcmp('SysGenIndex',get_param(bdroot(tmp_gcbh),'tag')) && ~isempty(regexp(bdroot(tmp_gcb), '^xbs', 'once')))
      |     return;
      |   end;
      |   xlMungeMaskParams;
      | 
      |   block_type='resource_estimator';
      | 
      |   serialized_declarations = '{''block_type''=>''String''}';
      |   xlresource_estimator_init();
      |   ptable_ = xlblockprep(get_param(tmp_gcb, 'MaskWSVariables'));
      |   try
      |     xlBlockMoveCallback(tmp_gcbh);
      |   catch 
      |      clear global xl_updateicon_recursion_guard;
      |   end;
      | catch
      |   global dbgsysgen;
      |   if(~isempty(dbgsysgen) && dbgsysgen)
      |     e = regexprep(lasterr, '\n', '\nError: ');
      |     disp(['Error: While running MaskInit code on block ' tmp_gcb ': ' e]);
      |     error(e);
      |   end
      | end
      settings: AttributesFormatString=Resource\nEstimator  CopyFcn=xlBlockMoveCallback(gcbh);  DeleteFcn=xlDestroyGui(gcbh);  ModelCloseFcn=xlDestroyGui(gcbh);  PreSaveFcn=xlBlockPreSaveCallback(gcbh);  PostSaveFcn=xlBlockPostSaveCallback(gcbh);  DestroyFcn=xlDestroyGui(gcbh);  OpenFcn=xlOpenGui(gcbh, 'resource_estimator_gui.xml', @resourceestimatorenablement, @resourceestimatoraction)  CloseFcn=xlDestroyGui(gcbh);  MoveFcn=xlBlockMoveCallback(gcbh);
      mask Help: eval('');xlDoc('-book','sysgen','-topic','Resource_Estimator');
      mask StyleString: edit,edit,edit,edit,edit,edit,edit,edit,checkbox,edit,popup(Estimate|Quick|Post Map|Read Mrp),edit,edit,edit,edit,edit,edit,edit,edit,edit,edit,edit,edit
      mask Display:
      | fprintf('','COMMENT: begin icon graphics');
      | patch([0 53 53 0 0 ],[0 0 53 53 0 ],[1 1 1 ]);
      | plot([0 53 53 0 0 ],[0 0 53 53 0 ]);
      | patch([10.425 20.54 27.54 34.54 41.54 27.54 17.425 10.425 ],[33.77 33.77 40.77 33.77 40.77 40.77 40.77 33.77 ],[0.839 0.874 0.937 ]);
      | patch([17.425 27.54 20.54 10.425 17.425 ],[26.77 26.77 33.77 33.77 26.77 ],[0.77 0.82 0.91 ]);
      | patch([10.425 20.54 27.54 17.425 10.425 ],[19.77 19.77 26.77 26.77 19.77 ],[0.839 0.874 0.937 ]);
      | patch([17.425 41.54 34.54 27.54 20.54 10.425 17.425 ],[12.77 12.77 19.77 12.77 19.77 19.77 12.77 ],[0.77 0.82 0.91 ]);
      | fprintf('','COMMENT: end icon graphics');
      | fprintf('','COMMENT: begin icon text');
      | fprintf('','COMMENT: end icon text');
  Sample Time : S-Function  LoadFcn=xlBlockLoadCallback(gcbh);  FunctionName=sysgen  Parameters=ptable_  EnableBusSupport=off  mask(Xilinx Sample Time Block Block){infoedit=The Sample Time block reports the normalized sample period of its input.  A signal's normalized sample period is not equivalent to its Simulink absolute sample period.<br><br>Hardware notes: This block is implemented as a constant in hardware., has_advanced_control=0, sggui_pos=-1,-1,-1,-1, block_type=sampletime, block_version=, sg_icon_stat=30,32,1,1,white,blue,0,5d3f35fb,right,,[ ],[ ], sg_mask_display=|, sg_list_contents=, sg_blockgui_xml=}
      mask sg_mask_display=|
      | fprintf('','COMMENT: begin icon graphics');
      | patch([0 30 30 0 0 ],[0 0 32 32 0 ],[0.77 0.82 0.91 ]);
      | plot([0 30 30 0 0 ],[0 0 32 32 0 ]);
      | patch([6.1 11.88 15.88 19.88 23.88 15.88 10.1 6.1 ],[20.44 20.44 24.44 20.44 24.44 24.44 24.44 20.44 ],[1 1 1 ]);
      | patch([10.1 15.88 11.88 6.1 10.1 ],[16.44 16.44 20.44 20.44 16.44 ],[0.931 0.946 0.973 ]);
      | patch([6.1 11.88 15.88 10.1 6.1 ],[12.44 12.44 16.44 16.44 12.44 ],[1 1 1 ]);
      | patch([10.1 23.88 19.88 15.88 11.88 6.1 10.1 ],[8.44 8.44 12.44 8.44 12.44 12.44 8.44 ],[0.931 0.946 0.973 ]);
      | fprintf('','COMMENT: end icon graphics');
      | fprintf('','COMMENT: begin icon text');
      |
      |
      | color('black');disp('ST');
      | fprintf('','COMMENT: end icon text');
      mask prompts: infoedit ""; has_advanced_control ""; sggui_pos ""; block_type ""; block_version ""; sg_icon_stat ""; sg_mask_display ""; sg_list_contents ""; sg_blockgui_xml ""
      mask help:
      | The Sample Time block reports the normalized sample period of its input.  A signal's normalized sample period is not equivalent to its Simulink absolute sample period.
      |
      | Hardware notes: This block is implemented as a constant in hardware.
      mask init:
      | try
      |   tmp_gcb = gcb;
      |   tmp_gcbh = gcbh;
      |   if (strcmp('SysGenIndex',get_param(bdroot(tmp_gcbh),'tag')) && ~isempty(regexp(bdroot(tmp_gcb), '^xbs', 'once')))
      |     return;
      |   end;
      |   xlMungeMaskParams;
      |   block_config = 'sysgen_blockset:SampleTime_config';
      | 
      |   block_type='sampletime';
      | 
      |   serialized_declarations = '{''block_type''=>''String''}';
      |   ptable_ = xlblockprep(get_param(tmp_gcb, 'MaskWSVariables'));
      |   try
      |     xlBlockMoveCallback(tmp_gcbh);
      |   catch 
      |      clear global xl_updateicon_recursion_guard;
      |   end;
      | catch
      |   global dbgsysgen;
      |   if(~isempty(dbgsysgen) && dbgsysgen)
      |     e = regexprep(lasterr, '\n', '\nError: ');
      |     disp(['Error: While running MaskInit code on block ' tmp_gcb ': ' e]);
      |     error(e);
      |   end
      | end
      settings: CopyFcn=xlBlockMoveCallback(gcbh);  DeleteFcn=xlDestroyGui(gcbh);  ModelCloseFcn=xlDestroyGui(gcbh);  PreSaveFcn=xlBlockPreSaveCallback(gcbh);  PostSaveFcn=xlBlockPostSaveCallback(gcbh);  DestroyFcn=xlDestroyGui(gcbh);  OpenFcn=xlOpenGui(gcbh, 'sampletime_gui.xml', -1, -1)  CloseFcn=xlDestroyGui(gcbh);  MoveFcn=xlBlockMoveCallback(gcbh);
      mask Help: eval('');xlDoc('-book','sysgen','-topic','Sample_Time');
      mask Display:
      | fprintf('','COMMENT: begin icon graphics');
      | patch([0 30 30 0 0 ],[0 0 32 32 0 ],[0.77 0.82 0.91 ]);
      | plot([0 30 30 0 0 ],[0 0 32 32 0 ]);
      | patch([6.1 11.88 15.88 19.88 23.88 15.88 10.1 6.1 ],[20.44 20.44 24.44 20.44 24.44 24.44 24.44 20.44 ],[1 1 1 ]);
      | patch([10.1 15.88 11.88 6.1 10.1 ],[16.44 16.44 20.44 20.44 16.44 ],[0.931 0.946 0.973 ]);
      | patch([6.1 11.88 15.88 10.1 6.1 ],[12.44 12.44 16.44 16.44 12.44 ],[1 1 1 ]);
      | patch([10.1 23.88 19.88 15.88 11.88 6.1 10.1 ],[8.44 8.44 12.44 8.44 12.44 12.44 8.44 ],[0.931 0.946 0.973 ]);
      | fprintf('','COMMENT: end icon graphics');
      | fprintf('','COMMENT: begin icon text');
      | 
      | 
      | color('black');disp('ST');
      | fprintf('','COMMENT: end icon text');
  Scale : S-Function  LoadFcn=xlBlockLoadCallback(gcbh);  FunctionName=sysgen  Parameters=ptable_  EnableBusSupport=off  mask(Xilinx Input Scaler Block){infoedit=Scales input by a power of two by adjusting the binary point position.<br><br>Hardware notes: In hardware this block costs nothing., scale_factor=4, dbl_ovrd_sgadvanced=, dbl_ovrd=off, has_advanced_control=0, sggui_pos=-1,-1,-1,-1, block_type=scale, block_version=, sg_icon_stat=55,56,1,1,white,blue,0,b6a81430,right,,[ ],[ ], sg_mask_display=|, sg_list_contents=, sg_blockgui_xml=}
      mask sg_mask_display=|
      | fprintf('','COMMENT: begin icon graphics');
      | patch([0 55 55 0 0 ],[0 0 56 56 0 ],[0.77 0.82 0.91 ]);
      | plot([0 55 55 0 0 ],[0 0 56 56 0 ]);
      | patch([11.425 21.54 28.54 35.54 42.54 28.54 18.425 11.425 ],[35.77 35.77 42.77 35.77 42.77 42.77 42.77 35.77 ],[1 1 1 ]);
      | patch([18.425 28.54 21.54 11.425 18.425 ],[28.77 28.77 35.77 35.77 28.77 ],[0.931 0.946 0.973 ]);
      | patch([11.425 21.54 28.54 18.425 11.425 ],[21.77 21.77 28.77 28.77 21.77 ],[1 1 1 ]);
      | patch([18.425 42.54 35.54 28.54 21.54 11.425 18.425 ],[14.77 14.77 21.77 14.77 21.77 21.77 14.77 ],[0.931 0.946 0.973 ]);
      | fprintf('','COMMENT: end icon graphics');
      | fprintf('','COMMENT: begin icon text');
      |
      |
      | color('black');disp('\bf{2^{4}}','texmode','on');
      | fprintf('','COMMENT: end icon text');
      mask prompts: infoedit ""; scale_factor "Scale factor s (scale output by 2^s)"; dbl_ovrd_sgadvanced ""; dbl_ovrd "Override with doubles"; has_advanced_control ""; sggui_pos ""; block_type ""; block_version ""; sg_icon_stat ""; sg_mask_display ""; sg_list_contents ""; sg_blockgui_xml ""
      mask help:
      | Scales input by a power of two by adjusting the binary point position.
      |
      | Hardware notes: In hardware this block costs nothing.
      mask init:
      | try
      |   tmp_gcb = gcb;
      |   tmp_gcbh = gcbh;
      |   if (strcmp('SysGenIndex',get_param(bdroot(tmp_gcbh),'tag')) && ~isempty(regexp(bdroot(tmp_gcb), '^xbs', 'once')))
      |     return;
      |   end;
      |   xlMungeMaskParams;
      |   block_config = 'sysgen_blockset:Scale_config';
      | 
      |   block_type='scale';
      | 
      |   serialized_declarations = '{''dbl_ovrd''=>''Int'',''scale_factor''=>''Int'',''block_type''=>''String''}';
      |   xlscale_init();
      |   ptable_ = xlblockprep(get_param(tmp_gcb, 'MaskWSVariables'));
      |   try
      |     xlBlockMoveCallback(tmp_gcbh);
      |   catch 
      |      clear global xl_updateicon_recursion_guard;
      |   end;
      | catch
      |   global dbgsysgen;
      |   if(~isempty(dbgsysgen) && dbgsysgen)
      |     e = regexprep(lasterr, '\n', '\nError: ');
      |     disp(['Error: While running MaskInit code on block ' tmp_gcb ': ' e]);
      |     error(e);
      |   end
      | end
      settings: CopyFcn=xlBlockMoveCallback(gcbh);  DeleteFcn=xlDestroyGui(gcbh);  ModelCloseFcn=xlDestroyGui(gcbh);  PreSaveFcn=xlBlockPreSaveCallback(gcbh);  PostSaveFcn=xlBlockPostSaveCallback(gcbh);  DestroyFcn=xlDestroyGui(gcbh);  OpenFcn=xlOpenGui(gcbh, 'scale_gui.xml', @xlmagicenablement, -1)  CloseFcn=xlDestroyGui(gcbh);  MoveFcn=xlBlockMoveCallback(gcbh);
      mask Help: eval('');xlDoc('-book','sysgen','-topic','Scale');
      mask Display:
      | fprintf('','COMMENT: begin icon graphics');
      | patch([0 55 55 0 0 ],[0 0 56 56 0 ],[0.77 0.82 0.91 ]);
      | plot([0 55 55 0 0 ],[0 0 56 56 0 ]);
      | patch([11.425 21.54 28.54 35.54 42.54 28.54 18.425 11.425 ],[35.77 35.77 42.77 35.77 42.77 42.77 42.77 35.77 ],[1 1 1 ]);
      | patch([18.425 28.54 21.54 11.425 18.425 ],[28.77 28.77 35.77 35.77 28.77 ],[0.931 0.946 0.973 ]);
      | patch([11.425 21.54 28.54 18.425 11.425 ],[21.77 21.77 28.77 28.77 21.77 ],[1 1 1 ]);
      | patch([18.425 42.54 35.54 28.54 21.54 11.425 18.425 ],[14.77 14.77 21.77 14.77 21.77 21.77 14.77 ],[0.931 0.946 0.973 ]);
      | fprintf('','COMMENT: end icon graphics');
      | fprintf('','COMMENT: begin icon text');
      | 
      | 
      | color('black');disp('\bf{2^{4}}','texmode','on');
      | fprintf('','COMMENT: end icon text');
  Serial to Parallel : S-Function  LoadFcn=xlBlockLoadCallback(gcbh);  FunctionName=sysgen  Parameters=ptable_  EnableBusSupport=off  mask(Xilinx Serial to Parallel Converter Block){infoedit=Groups of samples presented serially at the input become single samples presented at the output., input_order_sgadvanced=, input_order=Least Significant Word First, arith_type_sgadvanced=, arith_type=Unsigned, output_bits=16, bin_pt=0, rst_sgadvanced=, rst=off, en_sgadvanced=, en=off, latency=1, dbl_ovrd_sgadvanced=, dbl_ovrd=off, xl_use_area_sgadvanced=, xl_use_area=off, xl_area=[0,0,0,0,0,0,0], input_bits=, has_advanced_control=0, sggui_pos=-1,-1,-1,-1, block_type=s2p, block_version=, sg_icon_stat=60,54,1,1,white,blue,0,fff27cbf,right,,[ ],[ ], sg_mask_display=|, sg_list_contents=, sg_blockgui_xml=}
      mask sg_mask_display=|
      | fprintf('','COMMENT: begin icon graphics');
      | patch([0 60 60 0 0 ],[0 0 54 54 0 ],[0.77 0.82 0.91 ]);
      | plot([0 60 60 0 0 ],[0 0 54 54 0 ]);
      | patch([14.425 24.54 31.54 38.54 45.54 31.54 21.425 14.425 ],[34.77 34.77 41.77 34.77 41.77 41.77 41.77 34.77 ],[1 1 1 ]);
      | patch([21.425 31.54 24.54 14.425 21.425 ],[27.77 27.77 34.77 34.77 27.77 ],[0.931 0.946 0.973 ]);
      | patch([14.425 24.54 31.54 21.425 14.425 ],[20.77 20.77 27.77 27.77 20.77 ],[1 1 1 ]);
      | patch([21.425 45.54 38.54 31.54 24.54 14.425 21.425 ],[13.77 13.77 20.77 13.77 20.77 20.77 13.77 ],[0.931 0.946 0.973 ]);
      | fprintf('','COMMENT: end icon graphics');
      | fprintf('','COMMENT: begin icon text');
      | color('black');port_label('input',1,'s');
      | color('black');port_label('output',1,'p');
      | color('black');disp('z^{-1}','texmode','on');
      | fprintf('','COMMENT: end icon text');
      mask prompts: infoedit ""; input_order_sgadvanced ""; input_order "Input order"; arith_type_sgadvanced ""; arith_type "Arithmetic type"; output_bits "Number of bits"; bin_pt "Binary point"; rst_sgadvanced ""; rst "Provide <tt>reset</tt> port"; en_sgadvanced ""; en "Provide <tt>enable</tt> port"; dbl_ovrd_sgadvanced ""; dbl_ovrd "Override with doubles"; xl_use_area_sgadvanced ""; xl_use_area "Define FPGA area for resource estimation"; xl_area "FPGA area [slices, FFs, BRAMs, LUTs, IOBs, emb. mults, TBUFs]"; input_bits ""; has_advanced_control ""; sggui_pos ""; block_type ""; block_version ""; sg_icon_stat ""; sg_mask_display ""; sg_list_contents ""; sg_blockgui_xml ""
      mask help: Groups of samples presented serially at the input become single samples presented at the output.
      mask init:
      | try
      |   tmp_gcb = gcb;
      |   tmp_gcbh = gcbh;
      |   if (strcmp('SysGenIndex',get_param(bdroot(tmp_gcbh),'tag')) && ~isempty(regexp(bdroot(tmp_gcb), '^xbs', 'once')))
      |     return;
      |   end;
      |   xlMungeMaskParams;
      |   block_config = 'sysgen_blockset:S2P_config';
      | 
      |   block_type='s2p';
      | 
      |   serialized_declarations = '{''arith_type''=>''Int'',''bin_pt''=>''Int'',''en''=>''Int'',''input_order''=>''Int'',''latency''=>''Int'',''output_bits''=>''Int'',''rst''=>''Bool'',''sim_engine''=>''Int'',''sysgen_root''=>''String'',''block_type''=>''String''}';
      |   xls2p_init();
      |   ptable_ = xlblockprep(get_param(tmp_gcb, 'MaskWSVariables'));
      |   try
      |     xlBlockMoveCallback(tmp_gcbh);
      |   catch 
      |      clear global xl_updateicon_recursion_guard;
      |   end;
      | catch
      |   global dbgsysgen;
      |   if(~isempty(dbgsysgen) && dbgsysgen)
      |     e = regexprep(lasterr, '\n', '\nError: ');
      |     disp(['Error: While running MaskInit code on block ' tmp_gcb ': ' e]);
      |     error(e);
      |   end
      | end
      settings: CopyFcn=xlBlockMoveCallback(gcbh);  DeleteFcn=xlDestroyGui(gcbh);  ModelCloseFcn=xlDestroyGui(gcbh);  PreSaveFcn=xlBlockPreSaveCallback(gcbh);  PostSaveFcn=xlBlockPostSaveCallback(gcbh);  DestroyFcn=xlDestroyGui(gcbh);  OpenFcn=xlOpenGui(gcbh, 's2p_gui.xml', @xlmagicenablement, -1)  CloseFcn=xlDestroyGui(gcbh);  MoveFcn=xlBlockMoveCallback(gcbh);
      mask Help: eval('');xlDoc('-book','sysgen','-topic','Serial_to_Parallel');
      mask StyleString: edit,edit,popup(Least Significant Word First|Most Significant Word First),edit,popup(Signed  (2's comp)|Unsigned),edit,edit,edit,checkbox,edit,checkbox,edit,edit,checkbox,edit,checkbox,edit,edit,edit,edit,edit,edit,edit,edit,edit,edit
      mask Display:
      | fprintf('','COMMENT: begin icon graphics');
      | patch([0 60 60 0 0 ],[0 0 54 54 0 ],[0.77 0.82 0.91 ]);
      | plot([0 60 60 0 0 ],[0 0 54 54 0 ]);
      | patch([14.425 24.54 31.54 38.54 45.54 31.54 21.425 14.425 ],[34.77 34.77 41.77 34.77 41.77 41.77 41.77 34.77 ],[1 1 1 ]);
      | patch([21.425 31.54 24.54 14.425 21.425 ],[27.77 27.77 34.77 34.77 27.77 ],[0.931 0.946 0.973 ]);
      | patch([14.425 24.54 31.54 21.425 14.425 ],[20.77 20.77 27.77 27.77 20.77 ],[1 1 1 ]);
      | patch([21.425 45.54 38.54 31.54 24.54 14.425 21.425 ],[13.77 13.77 20.77 13.77 20.77 20.77 13.77 ],[0.931 0.946 0.973 ]);
      | fprintf('','COMMENT: end icon graphics');
      | fprintf('','COMMENT: begin icon text');
      | color('black');port_label('input',1,'s');
      | color('black');port_label('output',1,'p');
      | color('black');disp('z^{-1}','texmode','on');
      | fprintf('','COMMENT: end icon text');
  Shared Memory : S-Function  LoadFcn=xlBlockLoadCallback(gcbh);  FunctionName=sysgen  Parameters=ptable_  EnableBusSupport=off  mask(Xilinx Shared Memory Random Access Memory Block){shared_memory_name='Bar', depth=16, ownership_sgadvanced=, ownership=Locally Owned and Initialized, initVector=sin(pi*(0:15)/16), en_sgadvanced=, en=off, mutex_sgadvanced=, mutex=Unprotected, mode_sgadvanced=, mode=Read and Write, write_mode_sgadvanced=, write_mode=Read After Write, time_out=0, latency=1, explicit_data_type_sgadvanced=, explicit_data_type=off, gui_display_data_type=Fixed-point, arith_type_sgadvanced=, arith_type=Signed  (2's comp), n_bits=16, bin_pt=14, preci_type_sgadvanced=, preci_type=Single, xl_use_area_sgadvanced=, xl_use_area=off, xl_area=[0,0,0,0,0,0,0], implementation=Block RAM, use_rpm=off, has_advanced_control=0, sggui_pos=-1,-1,-1,-1, block_type=shmem, block_version=, sg_icon_stat=80,90,3,1,white,blue,0,bf435243,right,,[ ],[ ], sg_mask_display=|, sg_list_contents=, sg_blockgui_xml=}
      mask sg_mask_display=|
      | fprintf('','COMMENT: begin icon graphics');
      | patch([0 80 80 0 0 ],[0 0 90 90 0 ],[0.77 0.82 0.91 ]);
      | plot([0 80 80 0 0 ],[0 0 90 90 0 ]);
      | patch([15.525 31.42 42.42 53.42 64.42 42.42 26.525 15.525 ],[57.21 57.21 68.21 57.21 68.21 68.21 68.21 57.21 ],[1 1 1 ]);
      | patch([26.525 42.42 31.42 15.525 26.525 ],[46.21 46.21 57.21 57.21 46.21 ],[0.931 0.946 0.973 ]);
      | patch([15.525 31.42 42.42 26.525 15.525 ],[35.21 35.21 46.21 46.21 35.21 ],[1 1 1 ]);
      | patch([26.525 64.42 53.42 42.42 31.42 15.525 26.525 ],[24.21 24.21 35.21 24.21 35.21 35.21 24.21 ],[0.931 0.946 0.973 ]);
      | fprintf('','COMMENT: end icon graphics');
      | fprintf('','COMMENT: begin icon text');
      | color('black');port_label('input',1,'addr');
      | color('black');port_label('input',2,'din');
      | color('black');port_label('input',3,'we');
      | color('black');port_label('output',1,'dout');
      | fprintf('','COMMENT: end icon text');
      mask prompts: shared_memory_name "Shared memory name"; ownership_sgadvanced ""; ownership "Ownership and initialization"; initVector "Initial value vector"; en_sgadvanced ""; en "Provide enable port"; mutex_sgadvanced ""; mutex "Access protection"; mode_sgadvanced ""; mode "Access mode"; write_mode_sgadvanced ""; write_mode "Write mode"; time_out "Memory access timeout (sec)"; explicit_data_type_sgadvanced ""; explicit_data_type "Specify explicit output type"; gui_display_data_type ""; arith_type_sgadvanced ""; arith_type "Arithmetic type"; n_bits "Number of bits"; bin_pt "Binary point"; preci_type_sgadvanced ""; preci_type ""; xl_use_area_sgadvanced ""; xl_use_area "Define FPGA area for resource estimation"; xl_area "FPGA area [slices, FFs, BRAMs, LUTs, IOBs, emb. mults, TBUFs]"; implementation ""; use_rpm ""; has_advanced_control ""; sggui_pos ""; block_type ""; block_version ""; sg_icon_stat ""; sg_mask_display ""; sg_list_contents ""; sg_blockgui_xml ""
      mask help: Xilinx Shared Memory Random Access Memory
      mask init:
      | try
      |   tmp_gcb = gcb;
      |   tmp_gcbh = gcbh;
      |   if (strcmp('SysGenIndex',get_param(bdroot(tmp_gcbh),'tag')) && ~isempty(regexp(bdroot(tmp_gcb), '^xbs', 'once')))
      |     return;
      |   end;
      |   xlMungeMaskParams;
      |   block_config = 'sysgen_blockset:shmem_config';
      | 
      |   block_type='shmem';
      | 
      |   serialized_declarations = '{''arith_type''=>''Int'',''bin_pt''=>''Int'',''dbl_ovrd''=>''Int'',''depth''=>''Int'',''en''=>''Int'',''explicit_data_type''=>''Int'',''gui_display_data_type''=>''Int'',''initVector''=>''DoubleVector'',''latency''=>''Int'',''mode''=>''Int'',''mutex''=>''Int'',''n_bits''=>''Int'',''ownership''=>''Int'',''preci_type''=>''Int'',''shared_memory_name''=>''String'',''time_out''=>''Double'',''write_mode''=>''Int'',''block_type''=>''String''}';
      |   ptable_ = xlblockprep(get_param(tmp_gcb, 'MaskWSVariables'));
      |   try
      |     xlBlockMoveCallback(tmp_gcbh);
      |   catch 
      |      clear global xl_updateicon_recursion_guard;
      |   end;
      | catch
      |   global dbgsysgen;
      |   if(~isempty(dbgsysgen) && dbgsysgen)
      |     e = regexprep(lasterr, '\n', '\nError: ');
      |     disp(['Error: While running MaskInit code on block ' tmp_gcb ': ' e]);
      |     error(e);
      |   end
      | end
      settings: AttributesFormatString=<< %<shared_memory_name> >>  CopyFcn=xlBlockMoveCallback(gcbh);  DeleteFcn=xlDestroyGui(gcbh);  ModelCloseFcn=xlDestroyGui(gcbh);  PreSaveFcn=xlBlockPreSaveCallback(gcbh);  PostSaveFcn=xlBlockPostSaveCallback(gcbh);  DestroyFcn=xlDestroyGui(gcbh);  OpenFcn=xlOpenGui(gcbh, 'shmem_gui.xml', @shmemenablement, @xlDatatypeAction)  CloseFcn=xlDestroyGui(gcbh);  MoveFcn=xlBlockMoveCallback(gcbh);
      mask Help: eval('');xlDoc('-book','sysgen','-topic','Shared_Memory');
      mask StyleString: edit,edit,edit,popup(Locally Owned and Initialized|Owned and Initialized Elsewhere),edit,edit,checkbox,edit,popup(Lockable|Unprotected),edit,popup(Read and Write|Read Only|Write Only),edit,popup(Read After Write|Read Before Write|No Read On Write),edit,edit,edit,checkbox,popup(Fixed-point|Floating-point),edit,popup(Signed  (2's comp)|Unsigned|Floating-point),edit,edit,edit,popup(Single),edit,checkbox,edit,edit,edit,edit,edit,edit,edit,edit,edit,edit,edit
      mask Display:
      | fprintf('','COMMENT: begin icon graphics');
      | patch([0 80 80 0 0 ],[0 0 90 90 0 ],[0.77 0.82 0.91 ]);
      | plot([0 80 80 0 0 ],[0 0 90 90 0 ]);
      | patch([15.525 31.42 42.42 53.42 64.42 42.42 26.525 15.525 ],[57.21 57.21 68.21 57.21 68.21 68.21 68.21 57.21 ],[1 1 1 ]);
      | patch([26.525 42.42 31.42 15.525 26.525 ],[46.21 46.21 57.21 57.21 46.21 ],[0.931 0.946 0.973 ]);
      | patch([15.525 31.42 42.42 26.525 15.525 ],[35.21 35.21 46.21 46.21 35.21 ],[1 1 1 ]);
      | patch([26.525 64.42 53.42 42.42 31.42 15.525 26.525 ],[24.21 24.21 35.21 24.21 35.21 35.21 24.21 ],[0.931 0.946 0.973 ]);
      | fprintf('','COMMENT: end icon graphics');
      | fprintf('','COMMENT: begin icon text');
      | color('black');port_label('input',1,'addr');
      | color('black');port_label('input',2,'din');
      | color('black');port_label('input',3,'we');
      | color('black');port_label('output',1,'dout');
      | fprintf('','COMMENT: end icon text');
  Shared Memory Read : S-Function  Priority=2  LoadFcn=xlBlockLoadCallback(gcbh);  FunctionName=xlfromshmem  Parameters=shmem_name,sample_time,outDims,isFrame,dataType,shmem_type  EnableBusSupport=off  mask(Xilinx Shared Memory Read Block){infoedit=Reads sequentially from a shared memory block., shmem_name='Bar', shmem_type_sgadvanced=, shmem_type=FIFO, sample_time=1, dataType_sgadvanced=, dataType=int8, outDims=[1 1], isFrame_sgadvanced=, isFrame=off, shmem_word=0, shmem_depth=0, has_advanced_control=0, sggui_pos=-1,-1,-1,-1, block_type=fromshmem, block_version=, sg_icon_stat=80,50,-1,-1,yellow,white,0,07734,right,,[ ],[ ], sg_mask_display=|, sg_list_contents=, sg_blockgui_xml=}
      mask sg_mask_display=|
      | fprintf('','COMMENT: begin icon graphics');
      | patch([0 80 80 0 0 ],[0 0 50 50 0 ],[1 1 1 ]);
      | plot([0 80 80 0 0 ],[0 0 50 50 0 ]);
      | patch([24.425 34.54 41.54 48.54 55.54 41.54 31.425 24.425 ],[32.77 32.77 39.77 32.77 39.77 39.77 39.77 32.77 ],[0.965 0.951 0.755 ]);
      | patch([31.425 41.54 34.54 24.425 31.425 ],[25.77 25.77 32.77 32.77 25.77 ],[0.95 0.93 0.65 ]);
      | patch([24.425 34.54 41.54 31.425 24.425 ],[18.77 18.77 25.77 25.77 18.77 ],[0.965 0.951 0.755 ]);
      | patch([31.425 55.54 48.54 41.54 34.54 24.425 31.425 ],[11.77 11.77 18.77 11.77 18.77 18.77 11.77 ],[0.95 0.93 0.65 ]);
      | fprintf('','COMMENT: end icon graphics');
      | fprintf('','COMMENT: begin icon text');
      | fprintf('','COMMENT: end icon text');port_label('output',1,'d');
      | fprintf('depth: %d\nwidth: %d',shmem_depth,shmem_word);
      mask prompts: infoedit ""; shmem_name "Shared memory name"; shmem_type_sgadvanced ""; shmem_type "Type"; sample_time "Sample time"; dataType_sgadvanced ""; dataType "Data type"; outDims "Output dimensions (N or [M,N])"; isFrame_sgadvanced ""; isFrame "Use frame-based output (otherwise sample-based)"; shmem_word ""; shmem_depth ""; has_advanced_control ""; sggui_pos ""; block_type ""; block_version ""; sg_icon_stat ""; sg_mask_display ""; sg_list_contents ""; sg_blockgui_xml ""
      mask help: Reads sequentially from a shared memory block.
      mask init:
      | try
      |   tmp_gcb = gcb;
      |   tmp_gcbh = gcbh;
      |   if (strcmp('SysGenIndex',get_param(bdroot(tmp_gcbh),'tag')) && ~isempty(regexp(bdroot(tmp_gcb), '^xbs', 'once')))
      |     return;
      |   end;
      |   xlMungeMaskParams;
      | 
      |   block_type='fromshmem';
      | 
      |   serialized_declarations = '{''block_type''=>''String''}';
      |   xlfromshmem_init();
      |   ptable_ = xlblockprep(get_param(tmp_gcb, 'MaskWSVariables'));
      |   try
      |     xlBlockMoveCallback(tmp_gcbh);
      |   catch 
      |      clear global xl_updateicon_recursion_guard;
      |   end;
      | catch
      |   global dbgsysgen;
      |   if(~isempty(dbgsysgen) && dbgsysgen)
      |     e = regexprep(lasterr, '\n', '\nError: ');
      |     disp(['Error: While running MaskInit code on block ' tmp_gcb ': ' e]);
      |     error(e);
      |   end
      | end
      settings: AttributesFormatString=<< %<shmem_name> >>  CopyFcn=xlBlockMoveCallback(gcbh);  DeleteFcn=xlDestroyGui(gcbh);  ModelCloseFcn=xlDestroyGui(gcbh);  PreSaveFcn=xlBlockPreSaveCallback(gcbh);  PostSaveFcn=xlBlockPostSaveCallback(gcbh);  DestroyFcn=xlDestroyGui(gcbh);  OpenFcn=xlOpenGui(gcbh, 'fromshmem_gui.xml', -1, -1)  CloseFcn=xlDestroyGui(gcbh);  MoveFcn=xlBlockMoveCallback(gcbh);
      mask Help: eval('');xlDoc('-book','sysgen','-topic','Shared_Memory_Read');
      mask StyleString: edit,edit,edit,popup(FIFO|Lockable memory),edit,edit,popup(int8|uint8|int16|uint16|int32|uint32),edit,edit,checkbox,edit,edit,edit,edit,edit,edit,edit,edit,edit,edit
      mask Display:
      | fprintf('','COMMENT: begin icon graphics');
      | patch([0 80 80 0 0 ],[0 0 50 50 0 ],[1 1 1 ]);
      | plot([0 80 80 0 0 ],[0 0 50 50 0 ]);
      | patch([24.425 34.54 41.54 48.54 55.54 41.54 31.425 24.425 ],[32.77 32.77 39.77 32.77 39.77 39.77 39.77 32.77 ],[0.965 0.951 0.755 ]);
      | patch([31.425 41.54 34.54 24.425 31.425 ],[25.77 25.77 32.77 32.77 25.77 ],[0.95 0.93 0.65 ]);
      | patch([24.425 34.54 41.54 31.425 24.425 ],[18.77 18.77 25.77 25.77 18.77 ],[0.965 0.951 0.755 ]);
      | patch([31.425 55.54 48.54 41.54 34.54 24.425 31.425 ],[11.77 11.77 18.77 11.77 18.77 18.77 11.77 ],[0.95 0.93 0.65 ]);
      | fprintf('','COMMENT: end icon graphics');
      | fprintf('','COMMENT: begin icon text');
      | fprintf('','COMMENT: end icon text');port_label('output',1,'d');
      | fprintf('depth: %d\nwidth: %d',shmem_depth,shmem_word);
  Shared Memory Write : S-Function  LoadFcn=xlBlockLoadCallback(gcbh);  FunctionName=xltoshmem  Parameters=shmem_name, shmem_type, skip_check  EnableBusSupport=off  mask(Xilinx Shared Memory Write Block){infoedit=Writes scalar, vector, matrix, or frame data into a shared memory., shmem_name='Bar', shmem_type_sgadvanced=, shmem_type=FIFO, skip_check=0, shmem_word=0, shmem_depth=0, has_advanced_control=0, sggui_pos=-1,-1,-1,-1, block_type=toshmem, block_version=, sg_icon_stat=80,52,-1,-1,yellow,white,0,07734,right,,[ ],[ ], sg_mask_display=|, sg_list_contents=, sg_blockgui_xml=}
      mask sg_mask_display=|
      | fprintf('','COMMENT: begin icon graphics');
      | patch([0 80 80 0 0 ],[0 0 52 52 0 ],[1 1 1 ]);
      | plot([0 80 80 0 0 ],[0 0 52 52 0 ]);
      | patch([24.425 34.54 41.54 48.54 55.54 41.54 31.425 24.425 ],[33.77 33.77 40.77 33.77 40.77 40.77 40.77 33.77 ],[0.965 0.951 0.755 ]);
      | patch([31.425 41.54 34.54 24.425 31.425 ],[26.77 26.77 33.77 33.77 26.77 ],[0.95 0.93 0.65 ]);
      | patch([24.425 34.54 41.54 31.425 24.425 ],[19.77 19.77 26.77 26.77 19.77 ],[0.965 0.951 0.755 ]);
      | patch([31.425 55.54 48.54 41.54 34.54 24.425 31.425 ],[12.77 12.77 19.77 12.77 19.77 19.77 12.77 ],[0.95 0.93 0.65 ]);
      | fprintf('','COMMENT: end icon graphics');
      | fprintf('','COMMENT: begin icon text');
      | fprintf('','COMMENT: end icon text');port_label('input',1,'d');
      | fprintf('depth: %d\nwidth: %d',shmem_depth,shmem_word);
      mask prompts: infoedit ""; shmem_name "Shared memory name"; shmem_type_sgadvanced ""; shmem_type "Type"; skip_check ""; shmem_word ""; shmem_depth ""; has_advanced_control ""; sggui_pos ""; block_type ""; block_version ""; sg_icon_stat ""; sg_mask_display ""; sg_list_contents ""; sg_blockgui_xml ""
      mask help: Writes scalar, vector, matrix, or frame data into a shared memory.
      mask init:
      | try
      |   tmp_gcb = gcb;
      |   tmp_gcbh = gcbh;
      |   if (strcmp('SysGenIndex',get_param(bdroot(tmp_gcbh),'tag')) && ~isempty(regexp(bdroot(tmp_gcb), '^xbs', 'once')))
      |     return;
      |   end;
      |   xlMungeMaskParams;
      | 
      |   block_type='toshmem';
      | 
      |   serialized_declarations = '{''block_type''=>''String''}';
      |   xltoshmem_init();
      |   ptable_ = xlblockprep(get_param(tmp_gcb, 'MaskWSVariables'));
      |   try
      |     xlBlockMoveCallback(tmp_gcbh);
      |   catch 
      |      clear global xl_updateicon_recursion_guard;
      |   end;
      | catch
      |   global dbgsysgen;
      |   if(~isempty(dbgsysgen) && dbgsysgen)
      |     e = regexprep(lasterr, '\n', '\nError: ');
      |     disp(['Error: While running MaskInit code on block ' tmp_gcb ': ' e]);
      |     error(e);
      |   end
      | end
      settings: AttributesFormatString=<< %<shmem_name> >>  CopyFcn=xlBlockMoveCallback(gcbh);  DeleteFcn=xlDestroyGui(gcbh);  ModelCloseFcn=xlDestroyGui(gcbh);  PreSaveFcn=xlBlockPreSaveCallback(gcbh);  PostSaveFcn=xlBlockPostSaveCallback(gcbh);  DestroyFcn=xlDestroyGui(gcbh);  OpenFcn=xlOpenGui(gcbh, 'toshmem_gui.xml', @toshmemenablement, -1)  CloseFcn=xlDestroyGui(gcbh);  MoveFcn=xlBlockMoveCallback(gcbh);
      mask Help: eval('');xlDoc('-book','sysgen','-topic','Shared_Memory_Write');
      mask StyleString: edit,edit,edit,popup(FIFO|Lockable memory),edit,edit,edit,edit,edit,edit,edit,edit,edit,edit,edit
      mask Display:
      | fprintf('','COMMENT: begin icon graphics');
      | patch([0 80 80 0 0 ],[0 0 52 52 0 ],[1 1 1 ]);
      | plot([0 80 80 0 0 ],[0 0 52 52 0 ]);
      | patch([24.425 34.54 41.54 48.54 55.54 41.54 31.425 24.425 ],[33.77 33.77 40.77 33.77 40.77 40.77 40.77 33.77 ],[0.965 0.951 0.755 ]);
      | patch([31.425 41.54 34.54 24.425 31.425 ],[26.77 26.77 33.77 33.77 26.77 ],[0.95 0.93 0.65 ]);
      | patch([24.425 34.54 41.54 31.425 24.425 ],[19.77 19.77 26.77 26.77 19.77 ],[0.965 0.951 0.755 ]);
      | patch([31.425 55.54 48.54 41.54 34.54 24.425 31.425 ],[12.77 12.77 19.77 12.77 19.77 19.77 12.77 ],[0.95 0.93 0.65 ]);
      | fprintf('','COMMENT: end icon graphics');
      | fprintf('','COMMENT: begin icon text');
      | fprintf('','COMMENT: end icon text');port_label('input',1,'d');
      | fprintf('depth: %d\nwidth: %d',shmem_depth,shmem_word);
  Shift : S-Function  LoadFcn=xlBlockLoadCallback(gcbh);  FunctionName=sysgen  Parameters=ptable_  EnableBusSupport=off  mask(Xilinx Binary Shift Operator Block){infoedit=Hardware notes: In hardware this block costs nothing if full output precision is used., shift_dir_sgadvanced=, shift_dir=Left, shift_bits=2, en_sgadvanced=, en=off, latency=0, precision_sgadvanced=, precision=Full, arith_type_sgadvanced=, arith_type=Signed  (2's comp), n_bits=16, bin_pt=14, quantization_sgadvanced=, quantization=Truncate, overflow_sgadvanced=, overflow=Wrap, dbl_ovrd_sgadvanced=, dbl_ovrd=off, xl_use_area_sgadvanced=, xl_use_area=off, xl_area=[0,0,0,0,0,0,0], has_advanced_control=0, sggui_pos=-1,-1,-1,-1, block_type=shift, block_version=, sg_icon_stat=60,56,1,1,white,blue,0,282f02ea,right,,[ ],[ ], sg_mask_display=|, sg_list_contents=, sg_blockgui_xml=}
      mask sg_mask_display=|
      | fprintf('','COMMENT: begin icon graphics');
      | patch([0 60 60 0 0 ],[0 0 56 56 0 ],[0.77 0.82 0.91 ]);
      | plot([0 60 60 0 0 ],[0 0 56 56 0 ]);
      | patch([12.2 23.76 31.76 39.76 47.76 31.76 20.2 12.2 ],[36.88 36.88 44.88 36.88 44.88 44.88 44.88 36.88 ],[1 1 1 ]);
      | patch([20.2 31.76 23.76 12.2 20.2 ],[28.88 28.88 36.88 36.88 28.88 ],[0.931 0.946 0.973 ]);
      | patch([12.2 23.76 31.76 20.2 12.2 ],[20.88 20.88 28.88 28.88 20.88 ],[1 1 1 ]);
      | patch([20.2 47.76 39.76 31.76 23.76 12.2 20.2 ],[12.88 12.88 20.88 12.88 20.88 20.88 12.88 ],[0.931 0.946 0.973 ]);
      | fprintf('','COMMENT: end icon graphics');
      | fprintf('','COMMENT: begin icon text');
      |
      |
      | color('black');disp('\bf{X << 2}','texmode','on');
      | fprintf('','COMMENT: end icon text');
      mask prompts: infoedit ""; shift_dir_sgadvanced ""; shift_dir "Shift direction"; shift_bits "Number of bits"; en_sgadvanced ""; en "Provide enable port"; precision_sgadvanced ""; arith_type_sgadvanced ""; arith_type "Output type"; n_bits "Number of bits"; bin_pt "Binary point"; quantization_sgadvanced ""; overflow_sgadvanced ""; dbl_ovrd_sgadvanced ""; dbl_ovrd "Override with doubles"; xl_use_area_sgadvanced ""; xl_use_area "Define FPGA area for resource estimation"; xl_area "FPGA area [slices, FFs, BRAMs, LUTs, IOBs, emb. mults, TBUFs]"; has_advanced_control ""; sggui_pos ""; block_type ""; block_version ""; sg_icon_stat ""; sg_mask_display ""; sg_list_contents ""; sg_blockgui_xml ""
      mask help: Hardware notes: In hardware this block costs nothing if full output precision is used.
      mask init:
      | try
      |   tmp_gcb = gcb;
      |   tmp_gcbh = gcbh;
      |   if (strcmp('SysGenIndex',get_param(bdroot(tmp_gcbh),'tag')) && ~isempty(regexp(bdroot(tmp_gcb), '^xbs', 'once')))
      |     return;
      |   end;
      |   xlMungeMaskParams;
      |   block_config = 'sysgen_blockset:Shift_config';
      | 
      |   block_type='shift';
      | 
      |   serialized_declarations = '{''arith_type''=>''Int'',''bin_pt''=>''Int'',''en''=>''Int'',''latency''=>''Int'',''n_bits''=>''Int'',''overflow''=>''Int'',''precision''=>''Int'',''quantization''=>''Int'',''shift_bits''=>''Int'',''shift_dir''=>''Int'',''block_type''=>''String''}';
      |   ptable_ = xlblockprep(get_param(tmp_gcb, 'MaskWSVariables'));
      |   try
      |     xlBlockMoveCallback(tmp_gcbh);
      |   catch 
      |      clear global xl_updateicon_recursion_guard;
      |   end;
      | catch
      |   global dbgsysgen;
      |   if(~isempty(dbgsysgen) && dbgsysgen)
      |     e = regexprep(lasterr, '\n', '\nError: ');
      |     disp(['Error: While running MaskInit code on block ' tmp_gcb ': ' e]);
      |     error(e);
      |   end
      | end
      settings: CopyFcn=xlBlockMoveCallback(gcbh);  DeleteFcn=xlDestroyGui(gcbh);  ModelCloseFcn=xlDestroyGui(gcbh);  PreSaveFcn=xlBlockPreSaveCallback(gcbh);  PostSaveFcn=xlBlockPostSaveCallback(gcbh);  DestroyFcn=xlDestroyGui(gcbh);  OpenFcn=xlOpenGui(gcbh, 'shift_gui.xml', @shiftenablement, -1)  CloseFcn=xlDestroyGui(gcbh);  MoveFcn=xlBlockMoveCallback(gcbh);
      mask Help: eval('');xlDoc('-book','sysgen','-topic','Shift');
      mask StyleString: edit,edit,popup(Left|Right),edit,edit,checkbox,edit,edit,popup(Full|User Defined),edit,popup(Signed  (2's comp)|Unsigned),edit,edit,edit,popup(Truncate|Round  (unbiased: +/- Inf)),edit,popup(Wrap|Saturate|Flag as error),edit,checkbox,edit,checkbox,edit,edit,edit,edit,edit,edit,edit,edit,edit
      mask Display:
      | fprintf('','COMMENT: begin icon graphics');
      | patch([0 60 60 0 0 ],[0 0 56 56 0 ],[0.77 0.82 0.91 ]);
      | plot([0 60 60 0 0 ],[0 0 56 56 0 ]);
      | patch([12.2 23.76 31.76 39.76 47.76 31.76 20.2 12.2 ],[36.88 36.88 44.88 36.88 44.88 44.88 44.88 36.88 ],[1 1 1 ]);
      | patch([20.2 31.76 23.76 12.2 20.2 ],[28.88 28.88 36.88 36.88 28.88 ],[0.931 0.946 0.973 ]);
      | patch([12.2 23.76 31.76 20.2 12.2 ],[20.88 20.88 28.88 28.88 20.88 ],[1 1 1 ]);
      | patch([20.2 47.76 39.76 31.76 23.76 12.2 20.2 ],[12.88 12.88 20.88 12.88 20.88 20.88 12.88 ],[0.931 0.946 0.973 ]);
      | fprintf('','COMMENT: end icon graphics');
      | fprintf('','COMMENT: begin icon text');
      | 
      | 
      | color('black');disp('\bf{X << 2}','texmode','on');
      | fprintf('','COMMENT: end icon text');
  Simulation Multiplexer : S-Function  LoadFcn=xlBlockLoadCallback(gcbh);  FunctionName=sysgen  Parameters=ptable_  EnableBusSupport=off  mask(Xilinx Simulation Multiplexer Block){infoedit=Distinguish input subsystems as "simulation only" and "generation only".  The input specified For Simulation will be used during Simulink simulation.  The input specified For Generation will be used during code generation.  This block will typically be used on the output of a HW Co-Simulation, Black Box, or ModelSim subsystem.<br><br>Hardware Notes: This block costs nothing., sim_sel=1, hw_sel=2, has_advanced_control=0, sggui_pos=-1,-1,-1,-1, block_type=simmux, block_version=, sg_icon_stat=50,51,2,1,white,blue,0,4170dd71,right,,[ ],[ ], sg_mask_display=|, sg_list_contents=, sg_blockgui_xml=}
      mask sg_mask_display=|
      | fprintf('','COMMENT: begin icon graphics');
      | patch([0 50 50 0 0 ],[0 0 51 51 0 ],[0.77 0.82 0.91 ]);
      | plot([0 50 50 0 0 ],[0 0 51 51 0 ]);
      | patch([9.425 19.54 26.54 33.54 40.54 26.54 16.425 9.425 ],[32.77 32.77 39.77 32.77 39.77 39.77 39.77 32.77 ],[1 1 1 ]);
      | patch([16.425 26.54 19.54 9.425 16.425 ],[25.77 25.77 32.77 32.77 25.77 ],[0.931 0.946 0.973 ]);
      | patch([9.425 19.54 26.54 16.425 9.425 ],[18.77 18.77 25.77 25.77 18.77 ],[1 1 1 ]);
      | patch([16.425 40.54 33.54 26.54 19.54 9.425 16.425 ],[11.77 11.77 18.77 11.77 18.77 18.77 11.77 ],[0.931 0.946 0.973 ]);
      | fprintf('','COMMENT: end icon graphics');
      | fprintf('','COMMENT: begin icon text');
      |
      |
      |
      | fprintf('','COMMENT: end icon text');color('red');
      | plot(swLineX,simSwLineY);
      | color('black');
      | plot(swLineX,hwSwLineY);
      mask prompts: infoedit ""; sim_sel "For simulation,  pass through data from input port:   (1 or 2)"; hw_sel "For generation,  pass through data from input port:   (1 or 2)"; has_advanced_control ""; sggui_pos ""; block_type ""; block_version ""; sg_icon_stat ""; sg_mask_display ""; sg_list_contents ""; sg_blockgui_xml ""
      mask help:
      | Distinguish input subsystems as "simulation only" and "generation only".  The input specified For Simulation will be used during Simulink simulation.  The input specified For Generation will be used during code generation.  This block will typically be used on the output of a HW Co-Simulation, Black Box, or ModelSim subsystem.
      |
      | Hardware Notes: This block costs nothing.
      mask init:
      | try
      |   tmp_gcb = gcb;
      |   tmp_gcbh = gcbh;
      |   xlMungeMaskParams;
      |   block_config = 'sysgen_blockset:SimMux_config';
      | 
      |   block_type='simmux';
      | 
      |   serialized_declarations = '{''hw_sel''=>''Int'',''period''=>''Double'',''sim_sel''=>''Int'',''block_type''=>''String''}';
      |   xlsimmux_init();
      |   ptable_ = xlblockprep(get_param(tmp_gcb, 'MaskWSVariables'));
      |   try
      |     xlBlockMoveCallback(tmp_gcbh);
      |   catch 
      |      clear global xl_updateicon_recursion_guard;
      |   end;
      | catch
      |   global dbgsysgen;
      |   if(~isempty(dbgsysgen) && dbgsysgen)
      |     e = regexprep(lasterr, '\n', '\nError: ');
      |     disp(['Error: While running MaskInit code on block ' tmp_gcb ': ' e]);
      |     error(e);
      |   end
      | end
      settings: CopyFcn=xlBlockMoveCallback(gcbh);  DeleteFcn=xlDestroyGui(gcbh);  ModelCloseFcn=xlDestroyGui(gcbh);  PreSaveFcn=xlBlockPreSaveCallback(gcbh);  PostSaveFcn=xlBlockPostSaveCallback(gcbh);  DestroyFcn=xlDestroyGui(gcbh);  OpenFcn=xlOpenGui(gcbh, 'simmux_gui.xml', -1, -1)  CloseFcn=xlDestroyGui(gcbh);  MoveFcn=xlBlockMoveCallback(gcbh);
      mask Help: eval('');xlDoc('-book','sysgen','-topic','Simulation_Multiplexer');
      mask Display:
      | fprintf('','COMMENT: begin icon graphics');
      | patch([0 50 50 0 0 ],[0 0 51 51 0 ],[0.77 0.82 0.91 ]);
      | plot([0 50 50 0 0 ],[0 0 51 51 0 ]);
      | patch([9.425 19.54 26.54 33.54 40.54 26.54 16.425 9.425 ],[32.77 32.77 39.77 32.77 39.77 39.77 39.77 32.77 ],[1 1 1 ]);
      | patch([16.425 26.54 19.54 9.425 16.425 ],[25.77 25.77 32.77 32.77 25.77 ],[0.931 0.946 0.973 ]);
      | patch([9.425 19.54 26.54 16.425 9.425 ],[18.77 18.77 25.77 25.77 18.77 ],[1 1 1 ]);
      | patch([16.425 40.54 33.54 26.54 19.54 9.425 16.425 ],[11.77 11.77 18.77 11.77 18.77 18.77 11.77 ],[0.931 0.946 0.973 ]);
      | fprintf('','COMMENT: end icon graphics');
      | fprintf('','COMMENT: begin icon text');
      | 
      | 
      | 
      | fprintf('','COMMENT: end icon text');color('red');
      | plot(swLineX,simSwLineY);
      | color('black');
      | plot(swLineX,hwSwLineY);
  SineCosine : S-Function  LoadFcn=xlBlockLoadCallback(gcbh);  FunctionName=sysgen  Parameters=ptable_  EnableBusSupport=off  mask(Xilinx Sine/Cosine Generator Block){mode_sgadvanced=, mode=Sine, neg_sin_sgadvanced=, neg_sin=off, neg_cos_sgadvanced=, neg_cos=off, n_bits=8, sym_output_sgadvanced=, sym_output=off, en_sgadvanced=, en=off, latency=2, dbl_ovrd_sgadvanced=, dbl_ovrd=off, explicit_period_sgadvanced=, explicit_period=off, period=1, mem_type_sgadvanced=, mem_type=Distributed Memory, pipeline_sgadvanced=, pipeline=off, use_rpm_sgadvanced=, use_rpm=on, xl_use_area_sgadvanced=, xl_use_area=off, xl_area=[0,0,0,0,0,0,0], useCore=, has_advanced_control=0, sggui_pos=-1,-1,-1,-1, block_type=sincos, block_version=, sg_icon_stat=55,34,-1,-1,white,blue,0,07734,right,,[ ],[ ], sg_mask_display=|, sg_list_contents=, sg_blockgui_xml=}
      mask sg_mask_display=|
      | fprintf('','COMMENT: begin icon graphics');
      | patch([0 55 55 0 0 ],[0 0 34 34 0 ],[0.77 0.82 0.91 ]);
      | plot([0 55 55 0 0 ],[0 0 34 34 0 ]);
      | patch([18.1 23.88 27.88 31.88 35.88 27.88 22.1 18.1 ],[21.44 21.44 25.44 21.44 25.44 25.44 25.44 21.44 ],[1 1 1 ]);
      | patch([22.1 27.88 23.88 18.1 22.1 ],[17.44 17.44 21.44 21.44 17.44 ],[0.931 0.946 0.973 ]);
      | patch([18.1 23.88 27.88 22.1 18.1 ],[13.44 13.44 17.44 17.44 13.44 ],[1 1 1 ]);
      | patch([22.1 35.88 31.88 27.88 23.88 18.1 22.1 ],[9.44 9.44 13.44 9.44 13.44 13.44 9.44 ],[0.931 0.946 0.973 ]);
      | fprintf('','COMMENT: end icon graphics');
      | fprintf('','COMMENT: begin icon text');
      | fprintf('','COMMENT: end icon text');
      mask prompts: mode_sgadvanced ""; mode "Function"; neg_sin_sgadvanced ""; neg_sin "Negative sine"; neg_cos_sgadvanced ""; neg_cos "Negative cosine"; n_bits "Output width"; sym_output_sgadvanced ""; sym_output "Symmetric output"; en_sgadvanced ""; en "Provide enable port"; dbl_ovrd_sgadvanced ""; dbl_ovrd "Override with doubles"; explicit_period_sgadvanced ""; explicit_period "Specify explicit sample period"; period ""; mem_type_sgadvanced ""; mem_type "Memory Type"; pipeline_sgadvanced ""; pipeline "Pipeline for maximum performance"; use_rpm_sgadvanced ""; use_rpm "Use pre-defined core placement information"; xl_use_area_sgadvanced ""; xl_use_area "Define FPGA area for resource estimation"; xl_area "FPGA area [slices, FFs, BRAMs, LUTs, IOBs, emb. mults, TBUFs]"; useCore ""; has_advanced_control ""; sggui_pos ""; block_type ""; block_version ""; sg_icon_stat ""; sg_mask_display ""; sg_list_contents ""; sg_blockgui_xml ""
      mask help: Xilinx Sine/Cosine Generator
      mask init:
      | try
      |   tmp_gcb = gcb;
      |   tmp_gcbh = gcbh;
      |   if (strcmp('SysGenIndex',get_param(bdroot(tmp_gcbh),'tag')) && ~isempty(regexp(bdroot(tmp_gcb), '^xbs', 'once')))
      |     return;
      |   end;
      |   xlMungeMaskParams;
      |   block_config = 'sysgen_blockset:Removed_config';
      | 
      |   block_type='sincos';
      | nport = get_param(gcbh, 'ports');
      | nin = nport(1);
      | nout = nport(2);
      | 
      |   serialized_declarations = '{''en''=>''Int'',''latency''=>''Int'',''mem_type''=>''Int'',''mode''=>''Int'',''n_bits''=>''Int'',''neg_cos''=>''Int'',''neg_sin''=>''Int'',''period''=>''Double'',''pipeline''=>''Int'',''sym_output''=>''Int'',''use_rpm''=>''Int'',''block_type''=>''String'',''nin''=>''Double'',''nout''=>''Double''}';
      |   ptable_ = xlblockprep(get_param(tmp_gcb, 'MaskWSVariables'));
      |   try
      |     xlBlockMoveCallback(tmp_gcbh);
      |   catch 
      |      clear global xl_updateicon_recursion_guard;
      |   end;
      | catch
      |   global dbgsysgen;
      |   if(~isempty(dbgsysgen) && dbgsysgen)
      |     e = regexprep(lasterr, '\n', '\nError: ');
      |     disp(['Error: While running MaskInit code on block ' tmp_gcb ': ' e]);
      |     error(e);
      |   end
      | end
      settings: CopyFcn=xlBlockMoveCallback(gcbh);  DeleteFcn=xlDestroyGui(gcbh);  ModelCloseFcn=xlDestroyGui(gcbh);  PreSaveFcn=xlBlockPreSaveCallback(gcbh);  PostSaveFcn=xlBlockPostSaveCallback(gcbh);  DestroyFcn=xlDestroyGui(gcbh);  OpenFcn=xlOpenGui(gcbh, 'sincos_gui.xml', @xlremovedenablement, -1)  CloseFcn=xlDestroyGui(gcbh);  MoveFcn=xlBlockMoveCallback(gcbh);
      mask Help: eval('');xlDoc('-book','sysgen','-topic','SineCosine');
      mask StyleString: edit,popup(Sine|Cosine|Sine and Cosine),edit,checkbox,edit,checkbox,edit,edit,checkbox,edit,checkbox,edit,edit,checkbox,edit,checkbox,edit,edit,popup(Distributed Memory|Block RAM),edit,checkbox,edit,checkbox,edit,checkbox,edit,edit,edit,edit,edit,edit,edit,edit,edit,edit
      mask Display:
      | fprintf('','COMMENT: begin icon graphics');
      | patch([0 55 55 0 0 ],[0 0 34 34 0 ],[0.77 0.82 0.91 ]);
      | plot([0 55 55 0 0 ],[0 0 34 34 0 ]);
      | patch([18.1 23.88 27.88 31.88 35.88 27.88 22.1 18.1 ],[21.44 21.44 25.44 21.44 25.44 25.44 25.44 21.44 ],[1 1 1 ]);
      | patch([22.1 27.88 23.88 18.1 22.1 ],[17.44 17.44 21.44 21.44 17.44 ],[0.931 0.946 0.973 ]);
      | patch([18.1 23.88 27.88 22.1 18.1 ],[13.44 13.44 17.44 17.44 13.44 ],[1 1 1 ]);
      | patch([22.1 35.88 31.88 27.88 23.88 18.1 22.1 ],[9.44 9.44 13.44 9.44 13.44 13.44 9.44 ],[0.931 0.946 0.973 ]);
      | fprintf('','COMMENT: end icon graphics');
      | fprintf('','COMMENT: begin icon text');
      | fprintf('','COMMENT: end icon text');
  Single Port RAM : S-Function  LoadFcn=xlBlockLoadCallback(gcbh);  FunctionName=sysgen  Parameters=ptable_  EnableBusSupport=off  mask(Xilinx Single Port Random Access Memory Block){depth=16, initVector=sin(pi*(0:15)/16), distributed_mem_sgadvanced=, distributed_mem=Block RAM, write_mode_sgadvanced=, write_mode=Read After Write, rst_sgadvanced=, rst=off, init_reg=0, en_sgadvanced=, en=off, latency=1, dbl_ovrd_sgadvanced=, dbl_ovrd=off, optimize_sgadvanced=, optimize=Area, use_rpm_sgadvanced=, use_rpm=on, xl_use_area_sgadvanced=, xl_use_area=off, xl_area=[0,0,0,0,0,0,0], has_advanced_control=0, sggui_pos=-1,-1,-1,-1, block_type=spram, block_version=, sg_icon_stat=60,54,3,1,white,blue,0,afe23399,right,,[ ],[ ], sg_mask_display=|, sg_list_contents=, sg_blockgui_xml=}
      mask sg_mask_display=|
      | fprintf('','COMMENT: begin icon graphics');
      | patch([0 60 60 0 0 ],[0 0 54 54 0 ],[0.77 0.82 0.91 ]);
      | plot([0 60 60 0 0 ],[0 0 54 54 0 ]);
      | patch([14.425 24.54 31.54 38.54 45.54 31.54 21.425 14.425 ],[34.77 34.77 41.77 34.77 41.77 41.77 41.77 34.77 ],[1 1 1 ]);
      | patch([21.425 31.54 24.54 14.425 21.425 ],[27.77 27.77 34.77 34.77 27.77 ],[0.931 0.946 0.973 ]);
      | patch([14.425 24.54 31.54 21.425 14.425 ],[20.77 20.77 27.77 27.77 20.77 ],[1 1 1 ]);
      | patch([21.425 45.54 38.54 31.54 24.54 14.425 21.425 ],[13.77 13.77 20.77 13.77 20.77 20.77 13.77 ],[0.931 0.946 0.973 ]);
      | fprintf('','COMMENT: end icon graphics');
      | fprintf('','COMMENT: begin icon text');
      | color('black');port_label('input',1,'addr');
      | color('black');port_label('input',2,'data');
      | color('black');port_label('input',3,'we');
      |
      | color('black');disp('z^{-1}','texmode','on');
      | fprintf('','COMMENT: end icon text');
      mask prompts: initVector "Initial value vector"; distributed_mem_sgadvanced ""; distributed_mem "Memory Type"; write_mode_sgadvanced ""; write_mode "Write Mode"; rst_sgadvanced ""; rst "Provide reset port for output register"; init_reg "Initial value for output register"; en_sgadvanced ""; en "Provide enable port"; dbl_ovrd_sgadvanced ""; dbl_ovrd "Override with doubles"; optimize_sgadvanced ""; optimize "Optimize for"; use_rpm_sgadvanced ""; use_rpm "Use pre-defined core placement information"; xl_use_area_sgadvanced ""; xl_use_area "Define FPGA area for resource estimation"; xl_area "FPGA area [slices, FFs, BRAMs, LUTs, IOBs, emb. mults, TBUFs]"; has_advanced_control ""; sggui_pos ""; block_type ""; block_version ""; sg_icon_stat ""; sg_mask_display ""; sg_list_contents ""; sg_blockgui_xml ""
      mask help: Xilinx Single Port Random Access Memory
      mask init:
      | try
      |   tmp_gcb = gcb;
      |   tmp_gcbh = gcbh;
      |   if (strcmp('SysGenIndex',get_param(bdroot(tmp_gcbh),'tag')) && ~isempty(regexp(bdroot(tmp_gcb), '^xbs', 'once')))
      |     return;
      |   end;
      |   xlMungeMaskParams;
      |   block_config = 'sysgen_blockset:SPRAM_config';
      | 
      |   block_type='spram';
      | 
      |   serialized_declarations = '{''depth''=>''Int'',''distributed_mem''=>''Int'',''en''=>''Int'',''initVector''=>''DoubleVector'',''init_reg''=>''Double'',''latency''=>''Int'',''optimize''=>''Int'',''rst''=>''Int'',''use_rpm''=>''Int'',''write_mode''=>''Int'',''block_type''=>''String''}';
      |   xlspram_init();
      |   ptable_ = xlblockprep(get_param(tmp_gcb, 'MaskWSVariables'));
      |   try
      |     xlBlockMoveCallback(tmp_gcbh);
      |   catch 
      |      clear global xl_updateicon_recursion_guard;
      |   end;
      | catch
      |   global dbgsysgen;
      |   if(~isempty(dbgsysgen) && dbgsysgen)
      |     e = regexprep(lasterr, '\n', '\nError: ');
      |     disp(['Error: While running MaskInit code on block ' tmp_gcb ': ' e]);
      |     error(e);
      |   end
      | end
      settings: CopyFcn=xlBlockMoveCallback(gcbh);  DeleteFcn=xlDestroyGui(gcbh);  ModelCloseFcn=xlDestroyGui(gcbh);  PreSaveFcn=xlBlockPreSaveCallback(gcbh);  PostSaveFcn=xlBlockPostSaveCallback(gcbh);  DestroyFcn=xlDestroyGui(gcbh);  OpenFcn=xlOpenGui(gcbh, 'spram_gui.xml', @spramenablement, -1)  CloseFcn=xlDestroyGui(gcbh);  MoveFcn=xlBlockMoveCallback(gcbh);
      mask Help: eval('');xlDoc('-book','sysgen','-topic','Single_Port_RAM');
      mask StyleString: edit,edit,edit,popup(Distributed memory|Block RAM),edit,popup(Read After Write|Read Before Write|No Read On Write),edit,checkbox,edit,edit,checkbox,edit,edit,checkbox,edit,popup(Area|Speed|Power),edit,checkbox,edit,checkbox,edit,edit,edit,edit,edit,edit,edit,edit,edit
      mask Display:
      | fprintf('','COMMENT: begin icon graphics');
      | patch([0 60 60 0 0 ],[0 0 54 54 0 ],[0.77 0.82 0.91 ]);
      | plot([0 60 60 0 0 ],[0 0 54 54 0 ]);
      | patch([14.425 24.54 31.54 38.54 45.54 31.54 21.425 14.425 ],[34.77 34.77 41.77 34.77 41.77 41.77 41.77 34.77 ],[1 1 1 ]);
      | patch([21.425 31.54 24.54 14.425 21.425 ],[27.77 27.77 34.77 34.77 27.77 ],[0.931 0.946 0.973 ]);
      | patch([14.425 24.54 31.54 21.425 14.425 ],[20.77 20.77 27.77 27.77 20.77 ],[1 1 1 ]);
      | patch([21.425 45.54 38.54 31.54 24.54 14.425 21.425 ],[13.77 13.77 20.77 13.77 20.77 20.77 13.77 ],[0.931 0.946 0.973 ]);
      | fprintf('','COMMENT: end icon graphics');
      | fprintf('','COMMENT: begin icon text');
      | color('black');port_label('input',1,'addr');
      | color('black');port_label('input',2,'data');
      | color('black');port_label('input',3,'we');
      | 
      | color('black');disp('z^{-1}','texmode','on');
      | fprintf('','COMMENT: end icon text');
  Single-Step Simulation : Subsystem  mask(Xilinx Single-Step Simulation. Block){infoedit=Single-Step\nSimulation, xl_status=Single-Step, xl_state=0, has_advanced_control=0, sggui_pos=-1,-1,-1,-1, block_type=single_step_simulation, block_version=, sg_icon_stat=64,48,-1,-1,blue,white,0,07734,right,,[ ],[ ], sg_mask_display=|, sg_list_contents=, sg_blockgui_xml=}
      mask sg_mask_display=|
      | fprintf('','COMMENT: begin icon graphics');
      | patch([0 64 64 0 0 ],[0 0 48 48 0 ],[1 1 1 ]);
      | plot([0 64 64 0 0 ],[0 0 48 48 0 ]);
      | patch([18.65 27.32 33.32 39.32 45.32 33.32 24.65 18.65 ],[30.66 30.66 36.66 30.66 36.66 36.66 36.66 30.66 ],[0.839 0.874 0.937 ]);
      | patch([24.65 33.32 27.32 18.65 24.65 ],[24.66 24.66 30.66 30.66 24.66 ],[0.77 0.82 0.91 ]);
      | patch([18.65 27.32 33.32 24.65 18.65 ],[18.66 18.66 24.66 24.66 18.66 ],[0.839 0.874 0.937 ]);
      | patch([24.65 45.32 39.32 33.32 27.32 18.65 24.65 ],[12.66 12.66 18.66 12.66 18.66 18.66 12.66 ],[0.77 0.82 0.91 ]);
      | fprintf('','COMMENT: end icon graphics');
      | fprintf('','COMMENT: begin icon text');
      | fprintf('','COMMENT: end icon text');fprintf('%s', xl_status);
      mask prompts: infoedit ""; xl_status ""; xl_state ""; has_advanced_control ""; sggui_pos ""; block_type ""; block_version ""; sg_icon_stat ""; sg_mask_display ""; sg_list_contents ""; sg_blockgui_xml ""
      mask help: Single-Step\nSimulation
      mask init:
      | try
      |   tmp_gcb = gcb;
      |   tmp_gcbh = gcbh;
      |   if (strcmp('SysGenIndex',get_param(bdroot(tmp_gcbh),'tag')) && ~isempty(regexp(bdroot(tmp_gcb), '^xbs', 'once')))
      |     return;
      |   end;
      |   xlMungeMaskParams;
      | 
      |   block_type='single_step_simulation';
      | 
      |   serialized_declarations = '{''block_type''=>''String''}';
      |   xlsingle_step_simulation_init();
      |   ptable_ = xlblockprep(get_param(tmp_gcb, 'MaskWSVariables'));
      |   try
      |     xlBlockMoveCallback(tmp_gcbh);
      |   catch 
      |      clear global xl_updateicon_recursion_guard;
      |   end;
      | catch
      |   global dbgsysgen;
      |   if(~isempty(dbgsysgen) && dbgsysgen)
      |     e = regexprep(lasterr, '\n', '\nError: ');
      |     disp(['Error: While running MaskInit code on block ' tmp_gcb ': ' e]);
      |     error(e);
      |   end
      | end
      settings: CopyFcn=xlBlockMoveCallback(gcbh);  MoveFcn=xlBlockMoveCallback(gcbh);
      settings: OpenFcn=|
      | sw = get_param(gcb,'xl_state');
      | if(sw == '0')
      | set_param(gcb,'xl_state','1');
      | set_param(gcb,'xl_status','Continuous');
      | else
      | set_param(gcb,'xl_state','0');
      | set_param(gcb,'xl_status','Single-Step');
      | end
      mask Help: eval('');xlDoc('-book','sysgen','-topic','Single_Step_Simulation');
      mask Display:
      | fprintf('','COMMENT: begin icon graphics');
      | patch([0 64 64 0 0 ],[0 0 48 48 0 ],[1 1 1 ]);
      | plot([0 64 64 0 0 ],[0 0 48 48 0 ]);
      | patch([18.65 27.32 33.32 39.32 45.32 33.32 24.65 18.65 ],[30.66 30.66 36.66 30.66 36.66 36.66 36.66 30.66 ],[0.839 0.874 0.937 ]);
      | patch([24.65 33.32 27.32 18.65 24.65 ],[24.66 24.66 30.66 30.66 24.66 ],[0.77 0.82 0.91 ]);
      | patch([18.65 27.32 33.32 24.65 18.65 ],[18.66 18.66 24.66 24.66 18.66 ],[0.839 0.874 0.937 ]);
      | patch([24.65 45.32 39.32 33.32 27.32 18.65 24.65 ],[12.66 12.66 18.66 12.66 18.66 18.66 12.66 ],[0.77 0.82 0.91 ]);
      | fprintf('','COMMENT: end icon graphics');
      | fprintf('','COMMENT: begin icon text');
      | fprintf('','COMMENT: end icon text');fprintf('%s', xl_status);
  Slice : S-Function  LoadFcn=xlBlockLoadCallback(gcbh);  FunctionName=sysgen  Parameters=ptable_  EnableBusSupport=off  mask(Xilinx Bit Slice Extractor Block){infoedit=Extracts a given range of bits from each input sample and presents it at the output.  The output type is ordinarily unsigned with binary point at zero, but can be Boolean when the slice is one bit wide.<br><br>Hardware notes: In hardware this block costs nothing., nbits=1, boolean_output_sgadvanced=, boolean_output=off, mode_sgadvanced=, mode=Upper Bit Location + Width, bit1=0, base1_sgadvanced=, base1=MSB of Input, bit0=0, base0_sgadvanced=, base0=LSB of Input, dbl_ovrd_sgadvanced=, dbl_ovrd=off, has_advanced_control=0, sggui_pos=-1,-1,-1,-1, block_type=slice, block_version=, sg_icon_stat=60,30,1,1,white,blue,0,1fd851a7,right,,[ ],[ ], sg_mask_display=|, sg_list_contents=, sg_blockgui_xml=}
      mask sg_mask_display=|
      | fprintf('','COMMENT: begin icon graphics');
      | patch([0 60 60 0 0 ],[0 0 30 30 0 ],[0.77 0.82 0.91 ]);
      | plot([0 60 60 0 0 ],[0 0 30 30 0 ]);
      | patch([21.1 26.88 30.88 34.88 38.88 30.88 25.1 21.1 ],[19.44 19.44 23.44 19.44 23.44 23.44 23.44 19.44 ],[1 1 1 ]);
      | patch([25.1 30.88 26.88 21.1 25.1 ],[15.44 15.44 19.44 19.44 15.44 ],[0.931 0.946 0.973 ]);
      | patch([21.1 26.88 30.88 25.1 21.1 ],[11.44 11.44 15.44 15.44 11.44 ],[1 1 1 ]);
      | patch([25.1 38.88 34.88 30.88 26.88 21.1 25.1 ],[7.44 7.44 11.44 7.44 11.44 11.44 7.44 ],[0.931 0.946 0.973 ]);
      | fprintf('','COMMENT: end icon graphics');
      | fprintf('','COMMENT: begin icon text');
      |
      | color('black');port_label('output',1,'[a:b]');
      | fprintf('','COMMENT: end icon text');
      mask prompts: infoedit ""; nbits "Width of slice (number of bits)"; boolean_output_sgadvanced ""; boolean_output "Boolean output"; mode_sgadvanced ""; mode "Specify range as"; bit1 "Offset of top bit"; base1_sgadvanced ""; base1 "Relative to"; bit0 "Offset of bottom bit"; base0_sgadvanced ""; base0 "Relative to"; dbl_ovrd_sgadvanced ""; dbl_ovrd "Override with doubles"; has_advanced_control ""; sggui_pos ""; block_type ""; block_version ""; sg_icon_stat ""; sg_mask_display ""; sg_list_contents ""; sg_blockgui_xml ""
      mask help:
      | Extracts a given range of bits from each input sample and presents it at the output.  The output type is ordinarily unsigned with binary point at zero, but can be Boolean when the slice is one bit wide.
      |
      | Hardware notes: In hardware this block costs nothing.
      mask init:
      | try
      |   tmp_gcb = gcb;
      |   tmp_gcbh = gcbh;
      |   if (strcmp('SysGenIndex',get_param(bdroot(tmp_gcbh),'tag')) && ~isempty(regexp(bdroot(tmp_gcb), '^xbs', 'once')))
      |     return;
      |   end;
      |   xlMungeMaskParams;
      |   block_config = 'sysgen_blockset:Slice_config';
      | 
      |   block_type='slice';
      | 
      |   serialized_declarations = '{''base0''=>''Int'',''base1''=>''Int'',''bit0''=>''Int'',''bit1''=>''Int'',''boolean_output''=>''Int'',''mode''=>''Int'',''nbits''=>''Int'',''sim_engine''=>''Int'',''sysgen_root''=>''String'',''block_type''=>''String''}';
      |   xlslice_init();
      |   ptable_ = xlblockprep(get_param(tmp_gcb, 'MaskWSVariables'));
      |   try
      |     xlBlockMoveCallback(tmp_gcbh);
      |   catch 
      |      clear global xl_updateicon_recursion_guard;
      |   end;
      | catch
      |   global dbgsysgen;
      |   if(~isempty(dbgsysgen) && dbgsysgen)
      |     e = regexprep(lasterr, '\n', '\nError: ');
      |     disp(['Error: While running MaskInit code on block ' tmp_gcb ': ' e]);
      |     error(e);
      |   end
      | end
      settings: CopyFcn=xlBlockMoveCallback(gcbh);  DeleteFcn=xlDestroyGui(gcbh);  ModelCloseFcn=xlDestroyGui(gcbh);  PreSaveFcn=xlBlockPreSaveCallback(gcbh);  PostSaveFcn=xlBlockPostSaveCallback(gcbh);  DestroyFcn=xlDestroyGui(gcbh);  OpenFcn=xlOpenGui(gcbh, 'slice_gui.xml', @sliceenablement, -1)  CloseFcn=xlDestroyGui(gcbh);  MoveFcn=xlBlockMoveCallback(gcbh);
      mask Help: eval('');xlDoc('-book','sysgen','-topic','Slice');
      mask StyleString: edit,edit,edit,checkbox,edit,popup(Two Bit Locations|Upper Bit Location + Width|Lower Bit Location + Width),edit,edit,popup(LSB of Input|Binary Point of Input|MSB of Input),edit,edit,popup(LSB of Input|Binary Point of Input|MSB of Input),edit,checkbox,edit,edit,edit,edit,edit,edit,edit,edit
      mask Display:
      | fprintf('','COMMENT: begin icon graphics');
      | patch([0 60 60 0 0 ],[0 0 30 30 0 ],[0.77 0.82 0.91 ]);
      | plot([0 60 60 0 0 ],[0 0 30 30 0 ]);
      | patch([21.1 26.88 30.88 34.88 38.88 30.88 25.1 21.1 ],[19.44 19.44 23.44 19.44 23.44 23.44 23.44 19.44 ],[1 1 1 ]);
      | patch([25.1 30.88 26.88 21.1 25.1 ],[15.44 15.44 19.44 19.44 15.44 ],[0.931 0.946 0.973 ]);
      | patch([21.1 26.88 30.88 25.1 21.1 ],[11.44 11.44 15.44 15.44 11.44 ],[1 1 1 ]);
      | patch([25.1 38.88 34.88 30.88 26.88 21.1 25.1 ],[7.44 7.44 11.44 7.44 11.44 11.44 7.44 ],[0.931 0.946 0.973 ]);
      | fprintf('','COMMENT: end icon graphics');
      | fprintf('','COMMENT: begin icon text');
      | 
      | color('black');port_label('output',1,'[a:b]');
      | fprintf('','COMMENT: end icon text');
  SquareRoot : S-Function  LoadFcn=xlBlockLoadCallback(gcbh);  FunctionName=sysgen  Parameters=ptable_  EnableBusSupport=off  mask(Xilinx Square-Root Block){infoedit=Blocking: Wait for data on all inputs, allow back-pressure.<br>NonBlocking: operate every cycle in which all inputs are valid, no back-pressure., flow_control=NonBlocking, axi_optimize_goal=Resources, latency=0, rate=1, has_a_tlast=off, has_a_tuser=off, en=off, has_result_tready=off, has_invalid_op=off, xl_use_area_sgadvanced=, xl_use_area=off, xl_area=[0,0,0,0,0,0,0], fpo_op_type=square_root, has_b_tlast=false, has_b_tuser=false, result_tlast_behv=1, has_underflow=false, has_overflow=false, has_divide_by_zero=false, has_advanced_control=0, sggui_pos=-1,-1,-1,-1, block_type=squareroot, block_version=, sg_icon_stat=55,54,1,1,white,blue,0,6ed2cfaf,right,,[ ],[ ], sg_mask_display=|, sg_list_contents=, sg_blockgui_xml=}
      mask sg_mask_display=|
      | fprintf('','COMMENT: begin icon graphics');
      | patch([0 55 55 0 0 ],[0 0 54 54 0 ],[0.77 0.82 0.91 ]);
      | plot([0 55 55 0 0 ],[0 0 54 54 0 ]);
      | patch([11.425 21.54 28.54 35.54 42.54 28.54 18.425 11.425 ],[34.77 34.77 41.77 34.77 41.77 41.77 41.77 34.77 ],[1 1 1 ]);
      | patch([18.425 28.54 21.54 11.425 18.425 ],[27.77 27.77 34.77 34.77 27.77 ],[0.931 0.946 0.973 ]);
      | patch([11.425 21.54 28.54 18.425 11.425 ],[20.77 20.77 27.77 27.77 20.77 ],[1 1 1 ]);
      | patch([18.425 42.54 35.54 28.54 21.54 11.425 18.425 ],[13.77 13.77 20.77 13.77 20.77 20.77 13.77 ],[0.931 0.946 0.973 ]);
      | fprintf('','COMMENT: end icon graphics');
      | fprintf('','COMMENT: begin icon text');
      | color('black');port_label('input',1,'a');
      | color('black');port_label('output',1,'op');
      | fprintf('','COMMENT: end icon text');
      mask prompts: infoedit ""; flow_control "Flow Control"; axi_optimize_goal "Optimize Goal"; rate "Cycles/operation"; has_a_tlast "Has TLAST"; has_a_tuser "Has TUSER"; en "Provide enable port"; has_result_tready "Has Result TREADY"; has_invalid_op "INVALID_OP"; xl_use_area_sgadvanced ""; xl_use_area "Define FPGA area for resource estimation"; xl_area "FPGA area [slices, FFs, BRAMs, LUTs, IOBs, emb. mults, TBUFs]"; fpo_op_type ""; has_b_tlast ""; has_b_tuser ""; result_tlast_behv ""; has_underflow ""; has_overflow ""; has_divide_by_zero ""; has_advanced_control ""; sggui_pos ""; block_type ""; block_version ""; sg_icon_stat ""; sg_mask_display ""; sg_list_contents ""; sg_blockgui_xml ""
      mask help:
      | Blocking: Wait for data on all inputs, allow back-pressure.
      | NonBlocking: operate every cycle in which all inputs are valid, no back-pressure.
      mask init:
      | try
      |   tmp_gcb = gcb;
      |   tmp_gcbh = gcbh;
      |   if (strcmp('SysGenIndex',get_param(bdroot(tmp_gcbh),'tag')) && ~isempty(regexp(bdroot(tmp_gcb), '^xbs', 'once')))
      |     return;
      |   end;
      |   xlMungeMaskParams;
      |   block_config = 'sysgen:FPOBlockDescriptor_config';
      | 
      |   block_type='squareroot';
      | 
      |   serialized_declarations = '{''axi_optimize_goal''=>''String'',''en''=>''Bool'',''flow_control''=>''String'',''fpo_op_type''=>''String'',''has_a_tlast''=>''Bool'',''has_a_tuser''=>''Bool'',''has_b_tlast''=>''Bool'',''has_b_tuser''=>''Bool'',''has_divide_by_zero''=>''Bool'',''has_invalid_op''=>''Bool'',''has_overflow''=>''Bool'',''has_result_tready''=>''Bool'',''has_underflow''=>''Bool'',''latency''=>''Int'',''rate''=>''Int'',''result_tlast_behv''=>''Int'',''block_type''=>''String''}';
      |   ptable_ = xlblockprep(get_param(tmp_gcb, 'MaskWSVariables'));
      |   try
      |     xlBlockMoveCallback(tmp_gcbh);
      |   catch 
      |      clear global xl_updateicon_recursion_guard;
      |   end;
      | catch
      |   global dbgsysgen;
      |   if(~isempty(dbgsysgen) && dbgsysgen)
      |     e = regexprep(lasterr, '\n', '\nError: ');
      |     disp(['Error: While running MaskInit code on block ' tmp_gcb ': ' e]);
      |     error(e);
      |   end
      | end
      settings: CopyFcn=xlBlockMoveCallback(gcbh);  DeleteFcn=xlDestroyGui(gcbh);  ModelCloseFcn=xlDestroyGui(gcbh);  PreSaveFcn=xlBlockPreSaveCallback(gcbh);  PostSaveFcn=xlBlockPostSaveCallback(gcbh);  DestroyFcn=xlDestroyGui(gcbh);  OpenFcn=xlOpenGui(gcbh, 'squareroot_gui.xml', @sqrootenablement, @sqrootaction)  CloseFcn=xlDestroyGui(gcbh);  MoveFcn=xlBlockMoveCallback(gcbh);
      mask Help: eval('');xlDoc('-book','sysgen','-topic','SquareRoot');
      mask StyleString: edit,popup(Blocking|NonBlocking),popup(Resources|Performance),edit,edit,checkbox,checkbox,checkbox,checkbox,checkbox,edit,checkbox,edit,edit,edit,edit,edit,edit,edit,edit,edit,edit,edit,edit,edit,edit,edit,edit
      mask Display:
      | fprintf('','COMMENT: begin icon graphics');
      | patch([0 55 55 0 0 ],[0 0 54 54 0 ],[0.77 0.82 0.91 ]);
      | plot([0 55 55 0 0 ],[0 0 54 54 0 ]);
      | patch([11.425 21.54 28.54 35.54 42.54 28.54 18.425 11.425 ],[34.77 34.77 41.77 34.77 41.77 41.77 41.77 34.77 ],[1 1 1 ]);
      | patch([18.425 28.54 21.54 11.425 18.425 ],[27.77 27.77 34.77 34.77 27.77 ],[0.931 0.946 0.973 ]);
      | patch([11.425 21.54 28.54 18.425 11.425 ],[20.77 20.77 27.77 27.77 20.77 ],[1 1 1 ]);
      | patch([18.425 42.54 35.54 28.54 21.54 11.425 18.425 ],[13.77 13.77 20.77 13.77 20.77 20.77 13.77 ],[0.931 0.946 0.973 ]);
      | fprintf('','COMMENT: end icon graphics');
      | fprintf('','COMMENT: begin icon text');
      | color('black');port_label('input',1,'a');
      | color('black');port_label('output',1,'op');
      | fprintf('','COMMENT: end icon text');
  Threshold : S-Function  LoadFcn=xlBlockLoadCallback(gcbh);  FunctionName=sysgen  Parameters=ptable_  EnableBusSupport=off  mask(Xilinx Threshold Block){infoedit=Presents -1 as output if input is negative; otherwise presents 1.  Output is a two bit signed number., en_sgadvanced=, en=off, latency=0, dbl_ovrd_sgadvanced=, dbl_ovrd=off, xl_use_area_sgadvanced=, xl_use_area=off, xl_area=[0,0,0,0,0,0,0], has_advanced_control=0, sggui_pos=-1,-1,-1,-1, block_type=sgn, block_version=, sg_icon_stat=55,54,1,1,white,blue,0,b5a17a5d,right,,[ ],[ ], sg_mask_display=|, sg_list_contents=, sg_blockgui_xml=}
      mask sg_mask_display=|
      | fprintf('','COMMENT: begin icon graphics');
      | patch([0 55 55 0 0 ],[0 0 54 54 0 ],[0.77 0.82 0.91 ]);
      | plot([0 55 55 0 0 ],[0 0 54 54 0 ]);
      | patch([11.425 21.54 28.54 35.54 42.54 28.54 18.425 11.425 ],[34.77 34.77 41.77 34.77 41.77 41.77 41.77 34.77 ],[1 1 1 ]);
      | patch([18.425 28.54 21.54 11.425 18.425 ],[27.77 27.77 34.77 34.77 27.77 ],[0.931 0.946 0.973 ]);
      | patch([11.425 21.54 28.54 18.425 11.425 ],[20.77 20.77 27.77 27.77 20.77 ],[1 1 1 ]);
      | patch([18.425 42.54 35.54 28.54 21.54 11.425 18.425 ],[13.77 13.77 20.77 13.77 20.77 20.77 13.77 ],[0.931 0.946 0.973 ]);
      | fprintf('','COMMENT: end icon graphics');
      | fprintf('','COMMENT: begin icon text');
      |
      | color('black');port_label('output',1,'sgn');
      | fprintf('','COMMENT: end icon text');
      mask prompts: infoedit ""; en_sgadvanced ""; en "Provide enable port"; dbl_ovrd_sgadvanced ""; dbl_ovrd "Override with doubles"; xl_use_area_sgadvanced ""; xl_use_area "Define FPGA area for resource estimation"; xl_area "FPGA area [slices, FFs, BRAMs, LUTs, IOBs, emb. mults, TBUFs]"; has_advanced_control ""; sggui_pos ""; block_type ""; block_version ""; sg_icon_stat ""; sg_mask_display ""; sg_list_contents ""; sg_blockgui_xml ""
      mask help: Presents -1 as output if input is negative; otherwise presents 1. Output is a two bit signed number.
      mask init:
      | try
      |   tmp_gcb = gcb;
      |   tmp_gcbh = gcbh;
      |   if (strcmp('SysGenIndex',get_param(bdroot(tmp_gcbh),'tag')) && ~isempty(regexp(bdroot(tmp_gcb), '^xbs', 'once')))
      |     return;
      |   end;
      |   xlMungeMaskParams;
      |   block_config = 'sysgen_blockset:Sgn_config';
      | 
      |   block_type='sgn';
      | 
      |   serialized_declarations = '{''dbl_ovrd''=>''Int'',''en''=>''Int'',''latency''=>''Int'',''sim_engine''=>''Int'',''sysgen_root''=>''String'',''block_type''=>''String''}';
      |   xlsgn_init();
      |   ptable_ = xlblockprep(get_param(tmp_gcb, 'MaskWSVariables'));
      |   try
      |     xlBlockMoveCallback(tmp_gcbh);
      |   catch 
      |      clear global xl_updateicon_recursion_guard;
      |   end;
      | catch
      |   global dbgsysgen;
      |   if(~isempty(dbgsysgen) && dbgsysgen)
      |     e = regexprep(lasterr, '\n', '\nError: ');
      |     disp(['Error: While running MaskInit code on block ' tmp_gcb ': ' e]);
      |     error(e);
      |   end
      | end
      settings: CopyFcn=xlBlockMoveCallback(gcbh);  DeleteFcn=xlDestroyGui(gcbh);  ModelCloseFcn=xlDestroyGui(gcbh);  PreSaveFcn=xlBlockPreSaveCallback(gcbh);  PostSaveFcn=xlBlockPostSaveCallback(gcbh);  DestroyFcn=xlDestroyGui(gcbh);  OpenFcn=xlOpenGui(gcbh, 'sgn_gui.xml', @xlmagicenablement, -1)  CloseFcn=xlDestroyGui(gcbh);  MoveFcn=xlBlockMoveCallback(gcbh);
      mask Help: eval('');xlDoc('-book','sysgen','-topic','Threshold');
      mask Display:
      | fprintf('','COMMENT: begin icon graphics');
      | patch([0 55 55 0 0 ],[0 0 54 54 0 ],[0.77 0.82 0.91 ]);
      | plot([0 55 55 0 0 ],[0 0 54 54 0 ]);
      | patch([11.425 21.54 28.54 35.54 42.54 28.54 18.425 11.425 ],[34.77 34.77 41.77 34.77 41.77 41.77 41.77 34.77 ],[1 1 1 ]);
      | patch([18.425 28.54 21.54 11.425 18.425 ],[27.77 27.77 34.77 34.77 27.77 ],[0.931 0.946 0.973 ]);
      | patch([11.425 21.54 28.54 18.425 11.425 ],[20.77 20.77 27.77 27.77 20.77 ],[1 1 1 ]);
      | patch([18.425 42.54 35.54 28.54 21.54 11.425 18.425 ],[13.77 13.77 20.77 13.77 20.77 20.77 13.77 ],[0.931 0.946 0.973 ]);
      | fprintf('','COMMENT: end icon graphics');
      | fprintf('','COMMENT: begin icon text');
      | 
      | color('black');port_label('output',1,'sgn');
      | fprintf('','COMMENT: end icon text');
  Time Division Demultiplexer : S-Function  LoadFcn=xlBlockLoadCallback(gcbh);  FunctionName=sysgen  Parameters=ptable_  EnableBusSupport=off  mask(Xilinx Time Division Demultiplexer Block){infoedit=Samples presented at the input are selected and down-sampled according to the frame sampling pattern specified. The sampled input is presented either as a single or multiple channel at the output., frame_pattern=[1 1 1 1], impl_style_sgadvanced=, impl_style=Multiple Channel, vin_sgadvanced=, vin=off, dbl_ovrd_sgadvanced=, dbl_ovrd=off, xl_use_area_sgadvanced=, xl_use_area=off, xl_area=[0,0,0,0,0,0,0], explicit_period=off, period=1, has_advanced_control=0, sggui_pos=-1,-1,-1,-1, block_type=tdd, block_version=, sg_icon_stat=75,86,1,4,white,blue,0,8781f2a5,right,,[ ],[ ], sg_mask_display=|, sg_list_contents=, sg_blockgui_xml=}
      mask sg_mask_display=|
      | fprintf('','COMMENT: begin icon graphics');
      | patch([0 75 75 0 0 ],[0 0 86 86 0 ],[0.77 0.82 0.91 ]);
      | plot([0 75 75 0 0 ],[0 0 86 86 0 ]);
      | patch([14.75 29.2 39.2 49.2 59.2 39.2 24.75 14.75 ],[54.1 54.1 64.1 54.1 64.1 64.1 64.1 54.1 ],[1 1 1 ]);
      | patch([24.75 39.2 29.2 14.75 24.75 ],[44.1 44.1 54.1 54.1 44.1 ],[0.931 0.946 0.973 ]);
      | patch([14.75 29.2 39.2 24.75 14.75 ],[34.1 34.1 44.1 44.1 34.1 ],[1 1 1 ]);
      | patch([24.75 59.2 49.2 39.2 29.2 14.75 24.75 ],[24.1 24.1 34.1 24.1 34.1 34.1 24.1 ],[0.931 0.946 0.973 ]);
      | fprintf('','COMMENT: end icon graphics');
      | fprintf('','COMMENT: begin icon text');
      | color('black');port_label('input',1,'d');
      | color('black');port_label('output',1,'q0');
      | color('black');port_label('output',2,'q1');
      | color('black');port_label('output',3,'q2');
      | color('black');port_label('output',4,'q3');
      | color('black');disp('TDD');
      | fprintf('','COMMENT: end icon text');
      mask prompts: infoedit ""; frame_pattern "Frame sampling pattern (example: [1 0 1 0])"; impl_style_sgadvanced ""; impl_style "Implementation"; vin_sgadvanced ""; vin "Provide valid port"; dbl_ovrd_sgadvanced ""; dbl_ovrd "Override with doubles"; xl_use_area_sgadvanced ""; xl_use_area "Define FPGA area for resource estimation"; xl_area "FPGA area [slices, FFs, BRAMs, LUTs, IOBs, emb. mults, TBUFs]"; explicit_period ""; period ""; has_advanced_control ""; sggui_pos ""; block_type ""; block_version ""; sg_icon_stat ""; sg_mask_display ""; sg_list_contents ""; sg_blockgui_xml ""
      mask help: Samples presented at the input are selected and down-sampled according to the frame sampling pattern specified. The sampled input is presented either as a single or multiple channel at the output.
      mask init:
      | try
      |   tmp_gcb = gcb;
      |   tmp_gcbh = gcbh;
      |   if (strcmp('SysGenIndex',get_param(bdroot(tmp_gcbh),'tag')) && ~isempty(regexp(bdroot(tmp_gcb), '^xbs', 'once')))
      |     return;
      |   end;
      |   xlMungeMaskParams;
      |   block_config = 'sysgen_blockset:TDD_config';
      | 
      |   block_type='tdd';
      | 
      |   serialized_declarations = '{''frame_pattern''=>''String'',''impl_style''=>''Int'',''num_outputs''=>''Int'',''pattern''=>''IntVector'',''period''=>''Double'',''vin''=>''Int'',''block_type''=>''String''}';
      |   xltdd_init();
      |   ptable_ = xlblockprep(get_param(tmp_gcb, 'MaskWSVariables'));
      |   try
      |     xlBlockMoveCallback(tmp_gcbh);
      |   catch 
      |      clear global xl_updateicon_recursion_guard;
      |   end;
      | catch
      |   global dbgsysgen;
      |   if(~isempty(dbgsysgen) && dbgsysgen)
      |     e = regexprep(lasterr, '\n', '\nError: ');
      |     disp(['Error: While running MaskInit code on block ' tmp_gcb ': ' e]);
      |     error(e);
      |   end
      | end
      settings: CopyFcn=xlBlockMoveCallback(gcbh);  DeleteFcn=xlDestroyGui(gcbh);  ModelCloseFcn=xlDestroyGui(gcbh);  PreSaveFcn=xlBlockPreSaveCallback(gcbh);  PostSaveFcn=xlBlockPostSaveCallback(gcbh);  DestroyFcn=xlDestroyGui(gcbh);  OpenFcn=xlOpenGui(gcbh, 'tdd_gui.xml', @xlmagicenablement, -1)  CloseFcn=xlDestroyGui(gcbh);  MoveFcn=xlBlockMoveCallback(gcbh);
      mask Help: eval('');xlDoc('-book','sysgen','-topic','Time_Division_Demultiplexer');
      mask StyleString: edit,edit,edit,popup(Single Channel|Multiple Channel),edit,checkbox,edit,checkbox,edit,checkbox,edit,edit,edit,edit,edit,edit,edit,edit,edit,edit,edit
      mask Display:
      | fprintf('','COMMENT: begin icon graphics');
      | patch([0 75 75 0 0 ],[0 0 86 86 0 ],[0.77 0.82 0.91 ]);
      | plot([0 75 75 0 0 ],[0 0 86 86 0 ]);
      | patch([14.75 29.2 39.2 49.2 59.2 39.2 24.75 14.75 ],[54.1 54.1 64.1 54.1 64.1 64.1 64.1 54.1 ],[1 1 1 ]);
      | patch([24.75 39.2 29.2 14.75 24.75 ],[44.1 44.1 54.1 54.1 44.1 ],[0.931 0.946 0.973 ]);
      | patch([14.75 29.2 39.2 24.75 14.75 ],[34.1 34.1 44.1 44.1 34.1 ],[1 1 1 ]);
      | patch([24.75 59.2 49.2 39.2 29.2 14.75 24.75 ],[24.1 24.1 34.1 24.1 34.1 34.1 24.1 ],[0.931 0.946 0.973 ]);
      | fprintf('','COMMENT: end icon graphics');
      | fprintf('','COMMENT: begin icon text');
      | color('black');port_label('input',1,'d');
      | color('black');port_label('output',1,'q0');
      | color('black');port_label('output',2,'q1');
      | color('black');port_label('output',3,'q2');
      | color('black');port_label('output',4,'q3');
      | color('black');disp('TDD');
      | fprintf('','COMMENT: end icon text');
  Time Division Multiplexer : S-Function  LoadFcn=xlBlockLoadCallback(gcbh);  FunctionName=sysgen  Parameters=ptable_  EnableBusSupport=off  mask(Xilinx Time Division Multiplexer Block){infoedit=Multiple inputs are sampled and  presented serially at the output., inputs_sgadvanced=, inputs=4, vin_sgadvanced=, vin=off, dbl_ovrd_sgadvanced=, dbl_ovrd=off, xl_use_area_sgadvanced=, xl_use_area=off, xl_area=[0,0,0,0,0,0,0], explicit_period=off, period=1, has_advanced_control=0, sggui_pos=-1,-1,-1,-1, block_type=tdm, block_version=, sg_icon_stat=75,88,4,1,white,blue,0,4a8f92cb,right,,[ ],[ ], sg_mask_display=|, sg_list_contents=, sg_blockgui_xml=}
      mask sg_mask_display=|
      | fprintf('','COMMENT: begin icon graphics');
      | patch([0 75 75 0 0 ],[0 0 88 88 0 ],[0.77 0.82 0.91 ]);
      | plot([0 75 75 0 0 ],[0 0 88 88 0 ]);
      | patch([14.75 29.2 39.2 49.2 59.2 39.2 24.75 14.75 ],[55.1 55.1 65.1 55.1 65.1 65.1 65.1 55.1 ],[1 1 1 ]);
      | patch([24.75 39.2 29.2 14.75 24.75 ],[45.1 45.1 55.1 55.1 45.1 ],[0.931 0.946 0.973 ]);
      | patch([14.75 29.2 39.2 24.75 14.75 ],[35.1 35.1 45.1 45.1 35.1 ],[1 1 1 ]);
      | patch([24.75 59.2 49.2 39.2 29.2 14.75 24.75 ],[25.1 25.1 35.1 25.1 35.1 35.1 25.1 ],[0.931 0.946 0.973 ]);
      | fprintf('','COMMENT: end icon graphics');
      | fprintf('','COMMENT: begin icon text');
      | color('black');port_label('input',1,'d0');
      | color('black');port_label('input',2,'d1');
      | color('black');port_label('input',3,'d2');
      | color('black');port_label('input',4,'d3');
      | color('black');port_label('output',1,'q');
      | color('black');disp('TDM');
      | fprintf('','COMMENT: end icon text');
      mask prompts: infoedit ""; inputs_sgadvanced ""; inputs "Number of inputs"; vin_sgadvanced ""; vin "Provide valid port"; dbl_ovrd_sgadvanced ""; dbl_ovrd "Override with doubles"; xl_use_area_sgadvanced ""; xl_use_area "Define FPGA area for resource estimation"; xl_area "FPGA area [slices, FFs, BRAMs, LUTs, IOBs, emb. mults, TBUFs]"; explicit_period ""; period ""; has_advanced_control ""; sggui_pos ""; block_type ""; block_version ""; sg_icon_stat ""; sg_mask_display ""; sg_list_contents ""; sg_blockgui_xml ""
      mask help: Multiple inputs are sampled and presented serially at the output.
      mask init:
      | try
      |   tmp_gcb = gcb;
      |   tmp_gcbh = gcbh;
      |   if (strcmp('SysGenIndex',get_param(bdroot(tmp_gcbh),'tag')) && ~isempty(regexp(bdroot(tmp_gcb), '^xbs', 'once')))
      |     return;
      |   end;
      |   xlMungeMaskParams;
      |   block_config = 'sysgen_blockset:TDM_config';
      | 
      |   block_type='tdm';
      | 
      |   serialized_declarations = '{''inputs''=>''Int'',''vin''=>''Bool'',''block_type''=>''String''}';
      |   xltdm_init();
      |   ptable_ = xlblockprep(get_param(tmp_gcb, 'MaskWSVariables'));
      |   try
      |     xlBlockMoveCallback(tmp_gcbh);
      |   catch 
      |      clear global xl_updateicon_recursion_guard;
      |   end;
      | catch
      |   global dbgsysgen;
      |   if(~isempty(dbgsysgen) && dbgsysgen)
      |     e = regexprep(lasterr, '\n', '\nError: ');
      |     disp(['Error: While running MaskInit code on block ' tmp_gcb ': ' e]);
      |     error(e);
      |   end
      | end
      settings: CopyFcn=xlBlockMoveCallback(gcbh);  DeleteFcn=xlDestroyGui(gcbh);  ModelCloseFcn=xlDestroyGui(gcbh);  PreSaveFcn=xlBlockPreSaveCallback(gcbh);  PostSaveFcn=xlBlockPostSaveCallback(gcbh);  DestroyFcn=xlDestroyGui(gcbh);  OpenFcn=xlOpenGui(gcbh, 'tdm_gui.xml', @xlmagicenablement, -1)  CloseFcn=xlDestroyGui(gcbh);  MoveFcn=xlBlockMoveCallback(gcbh);
      mask Help: eval('');xlDoc('-book','sysgen','-topic','Time_Division_Multiplexer');
      mask StyleString: edit,edit,popup(2|3|4|5|6|7|8|9|10|11|12|13|14|15|16|17|18|19|20|21|22|23|24|25|26|27|28|29|30|31|32),edit,checkbox,edit,checkbox,edit,checkbox,edit,edit,edit,edit,edit,edit,edit,edit,edit,edit,edit
      mask Display:
      | fprintf('','COMMENT: begin icon graphics');
      | patch([0 75 75 0 0 ],[0 0 88 88 0 ],[0.77 0.82 0.91 ]);
      | plot([0 75 75 0 0 ],[0 0 88 88 0 ]);
      | patch([14.75 29.2 39.2 49.2 59.2 39.2 24.75 14.75 ],[55.1 55.1 65.1 55.1 65.1 65.1 65.1 55.1 ],[1 1 1 ]);
      | patch([24.75 39.2 29.2 14.75 24.75 ],[45.1 45.1 55.1 55.1 45.1 ],[0.931 0.946 0.973 ]);
      | patch([14.75 29.2 39.2 24.75 14.75 ],[35.1 35.1 45.1 45.1 35.1 ],[1 1 1 ]);
      | patch([24.75 59.2 49.2 39.2 29.2 14.75 24.75 ],[25.1 25.1 35.1 25.1 35.1 35.1 25.1 ],[0.931 0.946 0.973 ]);
      | fprintf('','COMMENT: end icon graphics');
      | fprintf('','COMMENT: begin icon text');
      | color('black');port_label('input',1,'d0');
      | color('black');port_label('input',2,'d1');
      | color('black');port_label('input',3,'d2');
      | color('black');port_label('input',4,'d3');
      | color('black');port_label('output',1,'q');
      | color('black');disp('TDM');
      | fprintf('','COMMENT: end icon text');
  To FIFO : S-Function  LoadFcn=xlBlockLoadCallback(gcbh);  FunctionName=sysgen  Parameters=ptable_  EnableBusSupport=off  mask(Xilinx Shared Memory Based To FIFO Block){infoedit=First-in-first-out (FIFO) block that writes FIFO data to shared memory storage., shared_memory_name='Bar', ownership_sgadvanced=, ownership=Locally owned, performance_options_sgadvanced=, performance_options=Standard_FIFO, depth_sgadvanced=, depth=16, percent_nbits_sgadvanced=, percent_nbits=1, has_arst_sgadvanced=, has_arst=off, use_percent_full_port_sgadvanced=, use_percent_full_port=on, explicit_data_type_sgadvanced=, explicit_data_type=off, gui_display_data_type=Fixed-point, arith_type_sgadvanced=, arith_type=Signed  (2's comp), n_bits=16, bin_pt=14, preci_type_sgadvanced=, preci_type=Single, dbl_ovrd_sgadvanced=, dbl_ovrd=off, mem_type_sgadvanced=, mem_type=Block RAM, xl_use_area_sgadvanced=, xl_use_area=off, xl_area=[0,0,0,0,0,0,0], has_advanced_control=0, sggui_pos=-1,-1,-1,-1, block_type=tofifo, block_version=, sg_icon_stat=80,91,2,2,white,blue,0,5474ed66,right,,[ ],[ ], sg_mask_display=|, sg_list_contents=, sg_blockgui_xml=}
      mask sg_mask_display=|
      | fprintf('','COMMENT: begin icon graphics');
      | patch([0 80 80 0 0 ],[0 0 91 91 0 ],[0.77 0.82 0.91 ]);
      | plot([0 80 80 0 0 ],[0 0 91 91 0 ]);
      | patch([15.525 31.42 42.42 53.42 64.42 42.42 26.525 15.525 ],[57.21 57.21 68.21 57.21 68.21 68.21 68.21 57.21 ],[1 1 1 ]);
      | patch([26.525 42.42 31.42 15.525 26.525 ],[46.21 46.21 57.21 57.21 46.21 ],[0.931 0.946 0.973 ]);
      | patch([15.525 31.42 42.42 26.525 15.525 ],[35.21 35.21 46.21 46.21 35.21 ],[1 1 1 ]);
      | patch([26.525 64.42 53.42 42.42 31.42 15.525 26.525 ],[24.21 24.21 35.21 24.21 35.21 35.21 24.21 ],[0.931 0.946 0.973 ]);
      | fprintf('','COMMENT: end icon graphics');
      | fprintf('','COMMENT: begin icon text');
      | color('black');port_label('input',1,'data_in');
      | color('black');port_label('input',2,'we');
      | color('black');port_label('output',1,'%full');
      | color('black');port_label('output',2,'full');
      | fprintf('','COMMENT: end icon text');
      mask prompts: infoedit ""; shared_memory_name "Shared memory name"; ownership_sgadvanced ""; performance_options_sgadvanced ""; performance_options "Performance Options"; depth_sgadvanced ""; percent_nbits_sgadvanced ""; percent_nbits "Bits of precision to use for <tt>%full</tt> port"; has_arst_sgadvanced ""; has_arst "Provide asynchronous reset port"; use_percent_full_port_sgadvanced ""; use_percent_full_port "Provide percent full port"; explicit_data_type_sgadvanced ""; explicit_data_type "Specify explicit output type"; gui_display_data_type ""; arith_type_sgadvanced ""; arith_type "Arithmetic type"; n_bits "Number of bits"; bin_pt "Binary point"; preci_type_sgadvanced ""; preci_type ""; dbl_ovrd_sgadvanced ""; dbl_ovrd "Override with doubles"; mem_type_sgadvanced ""; mem_type "Memory Type"; xl_use_area_sgadvanced ""; xl_use_area "Define FPGA area for resource estimation"; xl_area "FPGA area [slices, FFs, BRAMs, LUTs, IOBs, emb. mults, TBUFs]"; has_advanced_control ""; sggui_pos ""; block_type ""; block_version ""; sg_icon_stat ""; sg_mask_display ""; sg_list_contents ""; sg_blockgui_xml ""
      mask help: First-in-first-out (FIFO) block that writes FIFO data to shared memory storage.
      mask init:
      | try
      |   tmp_gcb = gcb;
      |   tmp_gcbh = gcbh;
      |   if (strcmp('SysGenIndex',get_param(bdroot(tmp_gcbh),'tag')) && ~isempty(regexp(bdroot(tmp_gcb), '^xbs', 'once')))
      |     return;
      |   end;
      |   xlMungeMaskParams;
      |   block_config = 'sysgen_blockset:tofifo_config';
      | 
      |   block_type='tofifo';
      | 
      |   serialized_declarations = '{''arith_type''=>''Int'',''bin_pt''=>''Int'',''dbl_ovrd''=>''Int'',''depth''=>''Int'',''explicit_data_type''=>''Int'',''gui_display_data_type''=>''Int'',''has_arst''=>''Int'',''mem_type''=>''Int'',''n_bits''=>''Int'',''ownership''=>''Int'',''percent_nbits''=>''Int'',''performance_options''=>''Int'',''preci_type''=>''Int'',''shared_memory_name''=>''String'',''use_percent_full_port''=>''Int'',''block_type''=>''String''}';
      |   ptable_ = xlblockprep(get_param(tmp_gcb, 'MaskWSVariables'));
      |   try
      |     xlBlockMoveCallback(tmp_gcbh);
      |   catch 
      |      clear global xl_updateicon_recursion_guard;
      |   end;
      | catch
      |   global dbgsysgen;
      |   if(~isempty(dbgsysgen) && dbgsysgen)
